simulink model "c00001M_harness"  (R2018a)
settings: Solver=ode3  StartTime=0.0  StopTime=10.0  RelTol=1e-3  EnableMultiTasking=on
undefined symbols (not defined in the file): b, DiscIntNeverNeededParam, J, K, L, R, sigbuilder_block
(part 3 of 19)

== system c00001M_harness/Eval66 ==
  In1 : Inport
  In2 : Inport  Port=2
  Constant3 : Constant
  Constant4 : Constant
  Data Type Conversion : DataTypeConversion
  Data Type Conversion1 : DataTypeConversion
  Memory1 : Memory  InitialCondition=1
  Memory2 : Memory  InitialCondition=1
  MinMax : MinMax  Inputs=4
  MinMax1 : MinMax  Inputs=2
  MinMax2 : MinMax  Inputs=2
  ROOut1 : RelationalOperator  Operator===  OutDataTypeStr=boolean  RndMeth=Simplest
  ROOut2 : RelationalOperator  Operator===  OutDataTypeStr=boolean  RndMeth=Simplest
  Out1 : Outport
  wires:
  Data Type Conversion1/1 -> MinMax2/1
  Data Type Conversion/1 -> MinMax1/1
  MinMax1/1 -> Memory1/1, MinMax/1
  MinMax2/1 -> Memory2/1, MinMax/2
  ROOut1/1 -> Data Type Conversion/1
  Memory2/1 -> MinMax2/2
  ROOut2/1 -> Data Type Conversion1/1
  Memory1/1 -> MinMax1/2
  [out2] -> ROOut2/2
  In1/1 -> ROOut1/1
  In2/1 -> ROOut2/1
  [out1] -> ROOut1/2
  MinMax/1 -> Out1/1
  Constant3/1 -> MinMax/3
  Constant4/1 -> MinMax/4

== system c00001M_harness/Eval67 ==
  In1 : Inport
  In2 : Inport  Port=2
  Constant3 : Constant
  Constant4 : Constant
  Data Type Conversion : DataTypeConversion
  Data Type Conversion1 : DataTypeConversion
  Memory1 : Memory  InitialCondition=1
  Memory2 : Memory  InitialCondition=1
  MinMax : MinMax  Inputs=4
  MinMax1 : MinMax  Inputs=2
  MinMax2 : MinMax  Inputs=2
  ROOut1 : RelationalOperator  Operator===  OutDataTypeStr=boolean  RndMeth=Simplest
  ROOut2 : RelationalOperator  Operator===  OutDataTypeStr=boolean  RndMeth=Simplest
  Out1 : Outport
  wires:
  Data Type Conversion1/1 -> MinMax2/1
  Data Type Conversion/1 -> MinMax1/1
  MinMax1/1 -> Memory1/1, MinMax/1
  MinMax2/1 -> Memory2/1, MinMax/2
  ROOut1/1 -> Data Type Conversion/1
  Memory2/1 -> MinMax2/2
  ROOut2/1 -> Data Type Conversion1/1
  Memory1/1 -> MinMax1/2
  [out2] -> ROOut2/2
  In1/1 -> ROOut1/1
  In2/1 -> ROOut2/1
  [out1] -> ROOut1/2
  MinMax/1 -> Out1/1
  Constant3/1 -> MinMax/3
  Constant4/1 -> MinMax/4

== system c00001M_harness/Eval70 ==
  In1 : Inport
  In2 : Inport  Port=2
  Constant3 : Constant
  Constant4 : Constant
  Data Type Conversion : DataTypeConversion
  Data Type Conversion1 : DataTypeConversion
  Memory1 : Memory  InitialCondition=1
  Memory2 : Memory  InitialCondition=1
  MinMax : MinMax  Inputs=4
  MinMax1 : MinMax  Inputs=2
  MinMax2 : MinMax  Inputs=2
  ROOut1 : RelationalOperator  Operator===  OutDataTypeStr=boolean  RndMeth=Simplest
  ROOut2 : RelationalOperator  Operator===  OutDataTypeStr=boolean  RndMeth=Simplest
  Out1 : Outport
  wires:
  Data Type Conversion1/1 -> MinMax2/1
  Data Type Conversion/1 -> MinMax1/1
  MinMax1/1 -> Memory1/1, MinMax/1
  MinMax2/1 -> Memory2/1, MinMax/2
  ROOut1/1 -> Data Type Conversion/1
  Memory2/1 -> MinMax2/2
  ROOut2/1 -> Data Type Conversion1/1
  Memory1/1 -> MinMax1/2
  [out2] -> ROOut2/2
  In1/1 -> ROOut1/1
  In2/1 -> ROOut2/1
  [out1] -> ROOut1/2
  MinMax/1 -> Out1/1
  Constant3/1 -> MinMax/3
  Constant4/1 -> MinMax/4

== system c00001M_harness/Eval71 ==
  In1 : Inport
  In2 : Inport  Port=2
  Constant3 : Constant
  Constant4 : Constant
  Data Type Conversion : DataTypeConversion
  Data Type Conversion1 : DataTypeConversion
  Memory1 : Memory  InitialCondition=1
  Memory2 : Memory  InitialCondition=1
  MinMax : MinMax  Inputs=4
  MinMax1 : MinMax  Inputs=2
  MinMax2 : MinMax  Inputs=2
  ROOut1 : RelationalOperator  Operator===  OutDataTypeStr=boolean  RndMeth=Simplest
  ROOut2 : RelationalOperator  Operator===  OutDataTypeStr=boolean  RndMeth=Simplest
  Out1 : Outport
  wires:
  Data Type Conversion1/1 -> MinMax2/1
  Data Type Conversion/1 -> MinMax1/1
  MinMax1/1 -> Memory1/1, MinMax/1
  MinMax2/1 -> Memory2/1, MinMax/2
  ROOut1/1 -> Data Type Conversion/1
  Memory2/1 -> MinMax2/2
  ROOut2/1 -> Data Type Conversion1/1
  Memory1/1 -> MinMax1/2
  [out2] -> ROOut2/2
  In1/1 -> ROOut1/1
  In2/1 -> ROOut2/1
  [out1] -> ROOut1/2
  MinMax/1 -> Out1/1
  Constant3/1 -> MinMax/3
  Constant4/1 -> MinMax/4

== system c00001M_harness/Eval74 ==
  In1 : Inport
  In2 : Inport  Port=2
  Constant3 : Constant
  Constant4 : Constant
  Data Type Conversion : DataTypeConversion
  Data Type Conversion1 : DataTypeConversion
  Memory1 : Memory  InitialCondition=1
  Memory2 : Memory  InitialCondition=1
  MinMax : MinMax  Inputs=4
  MinMax1 : MinMax  Inputs=2
  MinMax2 : MinMax  Inputs=2
  ROOut1 : RelationalOperator  Operator===  OutDataTypeStr=boolean  RndMeth=Simplest
  ROOut2 : RelationalOperator  Operator===  OutDataTypeStr=boolean  RndMeth=Simplest
  Out1 : Outport
  wires:
  Data Type Conversion1/1 -> MinMax2/1
  Data Type Conversion/1 -> MinMax1/1
  MinMax1/1 -> Memory1/1, MinMax/1
  MinMax2/1 -> Memory2/1, MinMax/2
  ROOut1/1 -> Data Type Conversion/1
  Memory2/1 -> MinMax2/2
  ROOut2/1 -> Data Type Conversion1/1
  Memory1/1 -> MinMax1/2
  [out2] -> ROOut2/2
  In1/1 -> ROOut1/1
  In2/1 -> ROOut2/1
  [out1] -> ROOut1/2
  MinMax/1 -> Out1/1
  Constant3/1 -> MinMax/3
  Constant4/1 -> MinMax/4

== system c00001M_harness/Eval75 ==
  In1 : Inport
  In2 : Inport  Port=2
  Constant3 : Constant
  Constant4 : Constant
  Data Type Conversion : DataTypeConversion
  Data Type Conversion1 : DataTypeConversion
  Memory1 : Memory  InitialCondition=1
  Memory2 : Memory  InitialCondition=1
  MinMax : MinMax  Inputs=4
  MinMax1 : MinMax  Inputs=2
  MinMax2 : MinMax  Inputs=2
  ROOut1 : RelationalOperator  Operator===  OutDataTypeStr=boolean  RndMeth=Simplest
  ROOut2 : RelationalOperator  Operator===  OutDataTypeStr=boolean  RndMeth=Simplest
  Out1 : Outport
  wires:
  Data Type Conversion1/1 -> MinMax2/1
  Data Type Conversion/1 -> MinMax1/1
  MinMax1/1 -> Memory1/1, MinMax/1
  MinMax2/1 -> Memory2/1, MinMax/2
  ROOut1/1 -> Data Type Conversion/1
  Memory2/1 -> MinMax2/2
  ROOut2/1 -> Data Type Conversion1/1
  Memory1/1 -> MinMax1/2
  [out2] -> ROOut2/2
  In1/1 -> ROOut1/1
  In2/1 -> ROOut2/1
  [out1] -> ROOut1/2
  MinMax/1 -> Out1/1
  Constant3/1 -> MinMax/3
  Constant4/1 -> MinMax/4

== system c00001M_harness/Eval78 ==
  In1 : Inport
  In2 : Inport  Port=2
  Constant3 : Constant
  Constant4 : Constant
  Data Type Conversion : DataTypeConversion
  Data Type Conversion1 : DataTypeConversion
  Memory1 : Memory  InitialCondition=1
  Memory2 : Memory  InitialCondition=1
  MinMax : MinMax  Inputs=4
  MinMax1 : MinMax  Inputs=2
  MinMax2 : MinMax  Inputs=2
  ROOut1 : RelationalOperator  Operator===  OutDataTypeStr=boolean  RndMeth=Simplest
  ROOut2 : RelationalOperator  Operator===  OutDataTypeStr=boolean  RndMeth=Simplest
  Out1 : Outport
  wires:
  Data Type Conversion1/1 -> MinMax2/1
  Data Type Conversion/1 -> MinMax1/1
  MinMax1/1 -> Memory1/1, MinMax/1
  MinMax2/1 -> Memory2/1, MinMax/2
  ROOut1/1 -> Data Type Conversion/1
  Memory2/1 -> MinMax2/2
  ROOut2/1 -> Data Type Conversion1/1
  Memory1/1 -> MinMax1/2
  [out2] -> ROOut2/2
  In1/1 -> ROOut1/1
  In2/1 -> ROOut2/1
  [out1] -> ROOut1/2
  MinMax/1 -> Out1/1
  Constant3/1 -> MinMax/3
  Constant4/1 -> MinMax/4

== system c00001M_harness/Eval79 ==
  In1 : Inport
  In2 : Inport  Port=2
  Constant3 : Constant
  Constant4 : Constant
  Data Type Conversion : DataTypeConversion
  Data Type Conversion1 : DataTypeConversion
  Memory1 : Memory  InitialCondition=1
  Memory2 : Memory  InitialCondition=1
  MinMax : MinMax  Inputs=4
  MinMax1 : MinMax  Inputs=2
  MinMax2 : MinMax  Inputs=2
  ROOut1 : RelationalOperator  Operator===  OutDataTypeStr=boolean  RndMeth=Simplest
  ROOut2 : RelationalOperator  Operator===  OutDataTypeStr=boolean  RndMeth=Simplest
  Out1 : Outport
  wires:
  Data Type Conversion1/1 -> MinMax2/1
  Data Type Conversion/1 -> MinMax1/1
  MinMax1/1 -> Memory1/1, MinMax/1
  MinMax2/1 -> Memory2/1, MinMax/2
  ROOut1/1 -> Data Type Conversion/1
  Memory2/1 -> MinMax2/2
  ROOut2/1 -> Data Type Conversion1/1
  Memory1/1 -> MinMax1/2
  [out2] -> ROOut2/2
  In1/1 -> ROOut1/1
  In2/1 -> ROOut2/1
  [out1] -> ROOut1/2
  MinMax/1 -> Out1/1
  Constant3/1 -> MinMax/3
  Constant4/1 -> MinMax/4

== system c00001M_harness/Eval82 ==
  In1 : Inport
  In2 : Inport  Port=2
  Constant3 : Constant
  Constant4 : Constant
  Data Type Conversion : DataTypeConversion
  Data Type Conversion1 : DataTypeConversion
  Memory1 : Memory  InitialCondition=1
  Memory2 : Memory  InitialCondition=1
  MinMax : MinMax  Inputs=4
  MinMax1 : MinMax  Inputs=2
  MinMax2 : MinMax  Inputs=2
  ROOut1 : RelationalOperator  Operator===  OutDataTypeStr=boolean  RndMeth=Simplest
  ROOut2 : RelationalOperator  Operator===  OutDataTypeStr=boolean  RndMeth=Simplest
  Out1 : Outport
  wires:
  Data Type Conversion1/1 -> MinMax2/1
  Data Type Conversion/1 -> MinMax1/1
  MinMax1/1 -> Memory1/1, MinMax/1
  MinMax2/1 -> Memory2/1, MinMax/2
  ROOut1/1 -> Data Type Conversion/1
  Memory2/1 -> MinMax2/2
  ROOut2/1 -> Data Type Conversion1/1
  Memory1/1 -> MinMax1/2
  [out2] -> ROOut2/2
  In1/1 -> ROOut1/1
  In2/1 -> ROOut2/1
  [out1] -> ROOut1/2
  MinMax/1 -> Out1/1
  Constant3/1 -> MinMax/3
  Constant4/1 -> MinMax/4

== system c00001M_harness/Eval83 ==
  In1 : Inport
  In2 : Inport  Port=2
  Constant3 : Constant
  Constant4 : Constant
  Data Type Conversion : DataTypeConversion
  Data Type Conversion1 : DataTypeConversion
  Memory1 : Memory  InitialCondition=1
  Memory2 : Memory  InitialCondition=1
  MinMax : MinMax  Inputs=4
  MinMax1 : MinMax  Inputs=2
  MinMax2 : MinMax  Inputs=2
  ROOut1 : RelationalOperator  Operator===  OutDataTypeStr=boolean  RndMeth=Simplest
  ROOut2 : RelationalOperator  Operator===  OutDataTypeStr=boolean  RndMeth=Simplest
  Out1 : Outport
  wires:
  Data Type Conversion1/1 -> MinMax2/1
  Data Type Conversion/1 -> MinMax1/1
  MinMax1/1 -> Memory1/1, MinMax/1
  MinMax2/1 -> Memory2/1, MinMax/2
  ROOut1/1 -> Data Type Conversion/1
  Memory2/1 -> MinMax2/2
  ROOut2/1 -> Data Type Conversion1/1
  Memory1/1 -> MinMax1/2
  [out2] -> ROOut2/2
  In1/1 -> ROOut1/1
  In2/1 -> ROOut2/1
  [out1] -> ROOut1/2
  MinMax/1 -> Out1/1
  Constant3/1 -> MinMax/3
  Constant4/1 -> MinMax/4

== system c00001M_harness/Eval86 ==
  In1 : Inport
  In2 : Inport  Port=2
  Constant3 : Constant
  Constant4 : Constant
  Data Type Conversion : DataTypeConversion
  Data Type Conversion1 : DataTypeConversion
  Memory1 : Memory  InitialCondition=1
  Memory2 : Memory  InitialCondition=1
  MinMax : MinMax  Inputs=4
  MinMax1 : MinMax  Inputs=2
  MinMax2 : MinMax  Inputs=2
  ROOut1 : RelationalOperator  Operator===  OutDataTypeStr=boolean  RndMeth=Simplest
  ROOut2 : RelationalOperator  Operator===  OutDataTypeStr=boolean  RndMeth=Simplest
  Out1 : Outport
  wires:
  Data Type Conversion1/1 -> MinMax2/1
  Data Type Conversion/1 -> MinMax1/1
  MinMax1/1 -> Memory1/1, MinMax/1
  MinMax2/1 -> Memory2/1, MinMax/2
  ROOut1/1 -> Data Type Conversion/1
  Memory2/1 -> MinMax2/2
  ROOut2/1 -> Data Type Conversion1/1
  Memory1/1 -> MinMax1/2
  [out2] -> ROOut2/2
  In1/1 -> ROOut1/1
  In2/1 -> ROOut2/1
  [out1] -> ROOut1/2
  MinMax/1 -> Out1/1
  Constant3/1 -> MinMax/3
  Constant4/1 -> MinMax/4

== system c00001M_harness/Eval87 ==
  In1 : Inport
  In2 : Inport  Port=2
  Constant3 : Constant
  Constant4 : Constant
  Data Type Conversion : DataTypeConversion
  Data Type Conversion1 : DataTypeConversion
  Memory1 : Memory  InitialCondition=1
  Memory2 : Memory  InitialCondition=1
  MinMax : MinMax  Inputs=4
  MinMax1 : MinMax  Inputs=2
  MinMax2 : MinMax  Inputs=2
  ROOut1 : RelationalOperator  Operator===  OutDataTypeStr=boolean  RndMeth=Simplest
  ROOut2 : RelationalOperator  Operator===  OutDataTypeStr=boolean  RndMeth=Simplest
  Out1 : Outport
  wires:
  Data Type Conversion1/1 -> MinMax2/1
  Data Type Conversion/1 -> MinMax1/1
  MinMax1/1 -> Memory1/1, MinMax/1
  MinMax2/1 -> Memory2/1, MinMax/2
  ROOut1/1 -> Data Type Conversion/1
  Memory2/1 -> MinMax2/2
  ROOut2/1 -> Data Type Conversion1/1
  Memory1/1 -> MinMax1/2
  [out2] -> ROOut2/2
  In1/1 -> ROOut1/1
  In2/1 -> ROOut2/1
  [out1] -> ROOut1/2
  MinMax/1 -> Out1/1
  Constant3/1 -> MinMax/3
  Constant4/1 -> MinMax/4

== system c00001M_harness/Eval90 ==
  In1 : Inport
  In2 : Inport  Port=2
  Constant3 : Constant
  Constant4 : Constant
  Data Type Conversion : DataTypeConversion
  Data Type Conversion1 : DataTypeConversion
  Memory1 : Memory  InitialCondition=1
  Memory2 : Memory  InitialCondition=1
  MinMax : MinMax  Inputs=4
  MinMax1 : MinMax  Inputs=2
  MinMax2 : MinMax  Inputs=2
  ROOut1 : RelationalOperator  Operator===  OutDataTypeStr=boolean  RndMeth=Simplest
  ROOut2 : RelationalOperator  Operator===  OutDataTypeStr=boolean  RndMeth=Simplest
  Out1 : Outport
  wires:
  Data Type Conversion1/1 -> MinMax2/1
  Data Type Conversion/1 -> MinMax1/1
  MinMax1/1 -> Memory1/1, MinMax/1
  MinMax2/1 -> Memory2/1, MinMax/2
  ROOut1/1 -> Data Type Conversion/1
  Memory2/1 -> MinMax2/2
  ROOut2/1 -> Data Type Conversion1/1
  Memory1/1 -> MinMax1/2
  [out2] -> ROOut2/2
  In1/1 -> ROOut1/1
  In2/1 -> ROOut2/1
  [out1] -> ROOut1/2
  MinMax/1 -> Out1/1
  Constant3/1 -> MinMax/3
  Constant4/1 -> MinMax/4

== system c00001M_harness/Eval91 ==
  In1 : Inport
  In2 : Inport  Port=2
  Constant3 : Constant
  Constant4 : Constant
  Data Type Conversion : DataTypeConversion
  Data Type Conversion1 : DataTypeConversion
  Memory1 : Memory  InitialCondition=1
  Memory2 : Memory  InitialCondition=1
  MinMax : MinMax  Inputs=4
  MinMax1 : MinMax  Inputs=2
  MinMax2 : MinMax  Inputs=2
  ROOut1 : RelationalOperator  Operator===  OutDataTypeStr=boolean  RndMeth=Simplest
  ROOut2 : RelationalOperator  Operator===  OutDataTypeStr=boolean  RndMeth=Simplest
  Out1 : Outport
  wires:
  Data Type Conversion1/1 -> MinMax2/1
  Data Type Conversion/1 -> MinMax1/1
  MinMax1/1 -> Memory1/1, MinMax/1
  MinMax2/1 -> Memory2/1, MinMax/2
  ROOut1/1 -> Data Type Conversion/1
  Memory2/1 -> MinMax2/2
  ROOut2/1 -> Data Type Conversion1/1
  Memory1/1 -> MinMax1/2
  [out2] -> ROOut2/2
  In1/1 -> ROOut1/1
  In2/1 -> ROOut2/1
  [out1] -> ROOut1/2
  MinMax/1 -> Out1/1
  Constant3/1 -> MinMax/3
  Constant4/1 -> MinMax/4

== system c00001M_harness/Eval94 ==
  In1 : Inport
  In2 : Inport  Port=2
  Constant3 : Constant
  Constant4 : Constant
  Data Type Conversion : DataTypeConversion
  Data Type Conversion1 : DataTypeConversion
  Memory1 : Memory  InitialCondition=1
  Memory2 : Memory  InitialCondition=1
  MinMax : MinMax  Inputs=4
  MinMax1 : MinMax  Inputs=2
  MinMax2 : MinMax  Inputs=2
  ROOut1 : RelationalOperator  Operator===  OutDataTypeStr=boolean  RndMeth=Simplest
  ROOut2 : RelationalOperator  Operator===  OutDataTypeStr=boolean  RndMeth=Simplest
  Out1 : Outport
  wires:
  Data Type Conversion1/1 -> MinMax2/1
  Data Type Conversion/1 -> MinMax1/1
  MinMax1/1 -> Memory1/1, MinMax/1
  MinMax2/1 -> Memory2/1, MinMax/2
  ROOut1/1 -> Data Type Conversion/1
  Memory2/1 -> MinMax2/2
  ROOut2/1 -> Data Type Conversion1/1
  Memory1/1 -> MinMax1/2
  [out2] -> ROOut2/2
  In1/1 -> ROOut1/1
  In2/1 -> ROOut2/1
  [out1] -> ROOut1/2
  MinMax/1 -> Out1/1
  Constant3/1 -> MinMax/3
  Constant4/1 -> MinMax/4

== system c00001M_harness/Eval95 ==
  In1 : Inport
  In2 : Inport  Port=2
  Constant3 : Constant
  Constant4 : Constant
  Data Type Conversion : DataTypeConversion
  Data Type Conversion1 : DataTypeConversion
  Memory1 : Memory  InitialCondition=1
  Memory2 : Memory  InitialCondition=1
  MinMax : MinMax  Inputs=4
  MinMax1 : MinMax  Inputs=2
  MinMax2 : MinMax  Inputs=2
  ROOut1 : RelationalOperator  Operator===  OutDataTypeStr=boolean  RndMeth=Simplest
  ROOut2 : RelationalOperator  Operator===  OutDataTypeStr=boolean  RndMeth=Simplest
  Out1 : Outport
  wires:
  Data Type Conversion1/1 -> MinMax2/1
  Data Type Conversion/1 -> MinMax1/1
  MinMax1/1 -> Memory1/1, MinMax/1
  MinMax2/1 -> Memory2/1, MinMax/2
  ROOut1/1 -> Data Type Conversion/1
  Memory2/1 -> MinMax2/2
  ROOut2/1 -> Data Type Conversion1/1
  Memory1/1 -> MinMax1/2
  [out2] -> ROOut2/2
  In1/1 -> ROOut1/1
  In2/1 -> ROOut2/1
  [out1] -> ROOut1/2
  MinMax/1 -> Out1/1
  Constant3/1 -> MinMax/3
  Constant4/1 -> MinMax/4

== system c00001M_harness/Eval98 ==
  In1 : Inport
  In2 : Inport  Port=2
  Constant3 : Constant
  Constant4 : Constant
  Data Type Conversion : DataTypeConversion
  Data Type Conversion1 : DataTypeConversion
  Memory1 : Memory  InitialCondition=1
  Memory2 : Memory  InitialCondition=1
  MinMax : MinMax  Inputs=4
  MinMax1 : MinMax  Inputs=2
  MinMax2 : MinMax  Inputs=2
  ROOut1 : RelationalOperator  Operator===  OutDataTypeStr=boolean  RndMeth=Simplest
  ROOut2 : RelationalOperator  Operator===  OutDataTypeStr=boolean  RndMeth=Simplest
  Out1 : Outport
  wires:
  Data Type Conversion1/1 -> MinMax2/1
  Data Type Conversion/1 -> MinMax1/1
  MinMax1/1 -> Memory1/1, MinMax/1
  MinMax2/1 -> Memory2/1, MinMax/2
  ROOut1/1 -> Data Type Conversion/1
  Memory2/1 -> MinMax2/2
  ROOut2/1 -> Data Type Conversion1/1
  Memory1/1 -> MinMax1/2
  [out2] -> ROOut2/2
  In1/1 -> ROOut1/1
  In2/1 -> ROOut2/1
  [out1] -> ROOut1/2
  MinMax/1 -> Out1/1
  Constant3/1 -> MinMax/3
  Constant4/1 -> MinMax/4

== system c00001M_harness/Eval99 ==
  In1 : Inport
  In2 : Inport  Port=2
  Constant3 : Constant
  Constant4 : Constant
  Data Type Conversion : DataTypeConversion
  Data Type Conversion1 : DataTypeConversion
  Memory1 : Memory  InitialCondition=1
  Memory2 : Memory  InitialCondition=1
  MinMax : MinMax  Inputs=4
  MinMax1 : MinMax  Inputs=2
  MinMax2 : MinMax  Inputs=2
  ROOut1 : RelationalOperator  Operator===  OutDataTypeStr=boolean  RndMeth=Simplest
  ROOut2 : RelationalOperator  Operator===  OutDataTypeStr=boolean  RndMeth=Simplest
  Out1 : Outport
  wires:
  Data Type Conversion1/1 -> MinMax2/1
  Data Type Conversion/1 -> MinMax1/1
  MinMax1/1 -> Memory1/1, MinMax/1
  MinMax2/1 -> Memory2/1, MinMax/2
  ROOut1/1 -> Data Type Conversion/1
  Memory2/1 -> MinMax2/2
  ROOut2/1 -> Data Type Conversion1/1
  Memory1/1 -> MinMax1/2
  [out2] -> ROOut2/2
  In1/1 -> ROOut1/1
  In2/1 -> ROOut2/1
  [out1] -> ROOut1/2
  MinMax/1 -> Out1/1
  Constant3/1 -> MinMax/3
  Constant4/1 -> MinMax/4

== system c00001M_harness/Inputs ==
  Demux : Demux  Tag=STV Demux
  FromWs : FromWorkspace  Tag=STV FromWs  VariableName=tuvar  SampleTime=0
      SigBuilderData=|
      | dataSet(1).timeRange = [0 20]
      | dataSet(1).name = 'Test Case 1'
      | dataSet(2).timeRange = [0 10]
      | dataSet(2).name = 'Test Case 2'
      | dataSet(3).timeRange = [0 8]
      | dataSet(3).name = 'Test Case 3'
      | dataSet(4).timeRange = [0 6]
      | dataSet(4).name = 'Test Case 4'
      | dataSet(5).timeRange = [0 6]
      | dataSet(5).name = 'Test Case 5'
      | dataSet(6).timeRange = [0 6]
      | dataSet(6).name = 'Test Case 6'
      | dataSet(7).timeRange = [0 8]
      | dataSet(7).name = 'Test Case 7'
      | dataSet(8).timeRange = [0 6]
      | dataSet(8).name = 'Test Case 8'
      | dataSet(9).timeRange = [0 6]
      | dataSet(9).name = 'Test Case 9'
      | dataSet(10).timeRange = [0 7]
      | dataSet(10).name = 'Test Case 10'
      | dataSet(11).timeRange = [0 9]
      | dataSet(11).name = 'Test Case 11'
      | dataSet(12).timeRange = [0 8]
      | dataSet(12).name = 'Test Case 12'
      | dataSet(13).timeRange = [0 12]
      | dataSet(13).name = 'Test Case 13'
      | dataSet(14).timeRange = [0 8]
      | dataSet(14).name = 'Test Case 14'
      | dataSet(15).timeRange = [0 8]
      | dataSet(15).name = 'Test Case 15'
      | dataSet(16).timeRange = [0 8]
      | dataSet(16).name = 'Test Case 16'
      | dataSet(17).timeRange = [0 8]
      | dataSet(17).name = 'Test Case 17'
      | dataSet(18).timeRange = [0 8]
      | dataSet(18).name = 'Test Case 18'
      | dataSet(19).timeRange = [0 8]
      | dataSet(19).name = 'Test Case 19'
      | dataSet(20).timeRange = [0 7]
      | dataSet(20).name = 'Test Case 20'
      | dataSet(21).timeRange = [0 7]
      | dataSet(21).name = 'Test Case 21'
      | dataSet(22).timeRange = [0 7]
      | dataSet(22).name = 'Test Case 22'
      | dataSet(23).timeRange = [0 8]
      | dataSet(23).name = 'Test Case 23'
      | dataSet(24).timeRange = [0 8]
      | dataSet(24).name = 'Test Case 24'
      | dataSet(25).timeRange = [0 8]
      | dataSet(25).name = 'Test Case 25'
      | dataSet(26).timeRange = [0 8]
      | dataSet(26).name = 'Test Case 26'
      | sbobj.Name = 'Signal Builder'
      | sbobj.Groups(1).Name = 'Test Case 1'
      | sbobj.Groups(1).Signals(1).Name = 'DW1'
      | sbobj.Groups(1).Signals(1).XData = [0 2 8 11 11 13 16 17 17 19 19 20]
      | sbobj.Groups(1).Signals(1).YData = [1 1 1 1 0 0 0 0 4 4 3 3]
      | sbobj.Groups(1).Signals(2).Name = 'P1W2'
      | sbobj.Groups(1).Signals(2).XData = [0 2 2 8 8 11 11 13 13 16 16 17 17 19 19 20]
      | sbobj.Groups(1).Signals(2).YData = [2 2 2 2 4 4 3 3 1 1 0 0 0 0 0 0]
      | sbobj.Groups(1).Signals(3).Name = 'O1'
      | sbobj.Groups(1).Signals(3).XData = [0 2 2 8 8 11 11 13 13 16 16 17 17 19 19 20]
      | sbobj.Groups(1).Signals(3).YData = [1 1 1 1 1 1 1 1 1 1 0 0 0 0 0 0]
      | sbobj.Groups(1).Signals(4).Name = 'O2'
      | sbobj.Groups(1).Signals(4).XData = [0 2 2 8 8 11 11 13 13 16 16 17 17 19 19 20]
      | sbobj.Groups(1).Signals(4).YData = [0 0 1 1 0 0 0 0 0 0 0 0 0 0 0 0]
      | sbobj.Groups(1).TimeRange = [0 20]
      | sbobj.Groups(2).Name = 'Test Case 2'
      | sbobj.Groups(2).Signals(1).Name = 'DW1'
      | sbobj.Groups(2).Signals(1).XData = [0 3 3 5 5 9 9 10]
      | sbobj.Groups(2).Signals(1).YData = [3 3 3 3 2 2 2 2]
      | sbobj.Groups(2).Signals(2).Name = 'P1W2'
      | sbobj.Groups(2).Signals(2).XData = [0 3 3 5 5 9 9 10]
      | sbobj.Groups(2).Signals(2).YData = [3 3 0 0 0 0 1 1]
      | sbobj.Groups(2).Signals(3).Name = 'O1'
      | sbobj.Groups(2).Signals(3).XData = [0 3 3 5 5 9 9 10]
      | sbobj.Groups(2).Signals(3).YData = [1 1 1 1 0 0 0 0]
      | sbobj.Groups(2).Signals(4).Name = 'O2'
      | sbobj.Groups(2).Signals(4).XData = [0 3 3 5 5 9 9 10]
      | sbobj.Groups(2).Signals(4).YData = [0 0 0 0 0 0 0 0]
      | sbobj.Groups(3).Name = 'Test Case 3'
      | sbobj.Groups(3).Signals(1).Name = 'DW1'
      | sbobj.Groups(3).Signals(1).XData = [0 3 3 4 4 7 7 8]
      | sbobj.Groups(3).Signals(1).YData = [4 4 0 0 1 1 1 1]
      | sbobj.Groups(3).Signals(2).Name = 'P1W2'
      | sbobj.Groups(3).Signals(2).XData = [0 3 3 4 4 7 7 8]
      | sbobj.Groups(3).Signals(2).YData = [4 4 1 1 0 0 3 3]
      | sbobj.Groups(3).Signals(3).Name = 'O1'
      | sbobj.Groups(3).Signals(3).XData = [0 3 3 4 4 7 7 8]
      | sbobj.Groups(3).Signals(3).YData = [0 0 0 0 0 0 0 0]
      | sbobj.Groups(3).Signals(4).Name = 'O2'
      | sbobj.Groups(3).Signals(4).XData = [0 3 3 4 4 7 7 8]
      | sbobj.Groups(3).Signals(4).YData = [0 0 0 0 0 0 0 0]
      | sbobj.Groups(3).TimeRange = [0 8]
      | sbobj.Groups(4).Name = 'Test Case 4'
      | sbobj.Groups(4).Signals(1).Name = 'DW1'
      | sbobj.Groups(4).Signals(1).XData = [0 3 3 5 5 6]
      | sbobj.Groups(4).Signals(1).YData = [4 4 2 2 2 2]
      | sbobj.Groups(4).Signals(2).Name = 'P1W2'
      | sbobj.Groups(4).Signals(2).XData = [0 3 3 5 5 6]
      | sbobj.Groups(4).Signals(2).YData = [1 1 0 0 0 0]
      | sbobj.Groups(4).Signals(3).Name = 'O1'
      | sbobj.Groups(4).Signals(3).XData = [0 3 3 5 5 6]
      | sbobj.Groups(4).Signals(3).YData = [0 0 0 0 0 0]
      | sbobj.Groups(4).Signals(4).Name = 'O2'
      | sbobj.Groups(4).Signals(4).XData = [0 3 3 5 5 6]
      | sbobj.Groups(4).Signals(4).YData = [0 0 0 0 1 1]
      | sbobj.Groups(4).TimeRange = [0 6]
      | sbobj.Groups(5).Name = 'Test Case 5'
      | sbobj.Groups(5).Signals(1).Name = 'DW1'
      | sbobj.Groups(5).Signals(1).XData = [0 3 3 5 5 6]
      | sbobj.Groups(5).Signals(1).YData = [3 3 0 0 3 3]
      | sbobj.Groups(5).Signals(2).Name = 'P1W2'
      | sbobj.Groups(5).Signals(2).XData = [0 3 3 5 5 6]
      | sbobj.Groups(5).Signals(2).YData = [4 4 0 0 3 3]
      | sbobj.Groups(5).Signals(3).Name = 'O1'
      | sbobj.Groups(5).Signals(3).XData = [0 3 3 5 5 6]
      | sbobj.Groups(5).Signals(3).YData = [0 0 0 0 1 1]
      | sbobj.Groups(5).Signals(4).Name = 'O2'
      | sbobj.Groups(5).Signals(4).XData = [0 3 3 5 5 6]
      | sbobj.Groups(5).Signals(4).YData = [1 1 0 0 0 0]
      | sbobj.Groups(5).TimeRange = [0 6]
      | sbobj.Groups(6).Name = 'Test Case 6'
      | sbobj.Groups(6).Signals(1).Name = 'DW1'
      | sbobj.Groups(6).Signals(1).XData = [0 3 3 5 5 6]
      | sbobj.Groups(6).Signals(1).YData = [1 1 1 1 0 0]
      | sbobj.Groups(6).Signals(2).Name = 'P1W2'
      | sbobj.Groups(6).Signals(2).XData = [0 3 3 5 5 6]
      | sbobj.Groups(6).Signals(2).YData = [4 4 2 2 0 0]
      | sbobj.Groups(6).Signals(3).Name = 'O1'
      | sbobj.Groups(6).Signals(3).XData = [0 3 3 5 5 6]
      | sbobj.Groups(6).Signals(3).YData = [1 1 1 1 1 1]
      | sbobj.Groups(6).Signals(4).Name = 'O2'
      | sbobj.Groups(6).Signals(4).XData = [0 3 3 5 5 6]
      | sbobj.Groups(6).Signals(4).YData = [0 0 0 0 1 1]
      | sbobj.Groups(6).TimeRange = [0 6]
      | sbobj.Groups(7).Name = 'Test Case 7'
      | sbobj.Groups(7).Signals(1).Name = 'DW1'
      | sbobj.Groups(7).Signals(1).XData = [0 3 3 4 4 7 7 8]
      | sbobj.Groups(7).Signals(1).YData = [1 1 1 1 1 1 3 3]
      | sbobj.Groups(7).Signals(2).Name = 'P1W2'
      | sbobj.Groups(7).Signals(2).XData = [0 3 3 4 4 7 7 8]
      | sbobj.Groups(7).Signals(2).YData = [4 4 3 3 2 2 0 0]
      | sbobj.Groups(7).Signals(3).Name = 'O1'
      | sbobj.Groups(7).Signals(3).XData = [0 3 3 4 4 7 7 8]
      | sbobj.Groups(7).Signals(3).YData = [1 1 1 1 1 1 0 0]
      | sbobj.Groups(7).Signals(4).Name = 'O2'
      | sbobj.Groups(7).Signals(4).XData = [0 3 3 4 4 7 7 8]
      | sbobj.Groups(7).Signals(4).YData = [0 0 0 0 0 0 1 1]
      | sbobj.Groups(7).TimeRange = [0 8]
      | sbobj.Groups(8).Name = 'Test Case 8'
      | sbobj.Groups(8).Signals(1).Name = 'DW1'
      | sbobj.Groups(8).Signals(1).XData = [0 2 2 3 3 5 5 6]
      | sbobj.Groups(8).Signals(1).YData = [1 1 2 2 2 2 2 2]
      | sbobj.Groups(8).Signals(2).Name = 'P1W2'
      | sbobj.Groups(8).Signals(2).XData = [0 2 2 3 3 5 5 6]
      | sbobj.Groups(8).Signals(2).YData = [4 4 3 3 1 1 3 3]
      | sbobj.Groups(8).Signals(3).Name = 'O1'
      | sbobj.Groups(8).Signals(3).XData = [0 2 2 3 3 5 5 6]
      | sbobj.Groups(8).Signals(3).YData = [1 1 1 1 1 1 0 0]
      | sbobj.Groups(8).Signals(4).Name = 'O2'
      | sbobj.Groups(8).Signals(4).XData = [0 2 2 3 3 5 5 6]
      | sbobj.Groups(8).Signals(4).YData = [0 0 1 1 0 0 0 0]
      | sbobj.Groups(8).TimeRange = [0 6]
      | sbobj.Groups(9).Name = 'Test Case 9'
      | sbobj.Groups(9).Signals(1).Name = 'DW1'
      | sbobj.Groups(9).Signals(1).XData = [0 2 2 3 3 5 5 6]
      | sbobj.Groups(9).Signals(1).YData = [1 1 4 4 3 3 2 2]
      | sbobj.Groups(9).Signals(2).Name = 'P1W2'
      | sbobj.Groups(9).Signals(2).XData = [0 2 2 3 3 5 5 6]
      | sbobj.Groups(9).Signals(2).YData = [4 4 0 0 0 0 1 1]
      | sbobj.Groups(9).Signals(3).Name = 'O1'
      | sbobj.Groups(9).Signals(3).XData = [0 2 2 3 3 5 5 6]
      | sbobj.Groups(9).Signals(3).YData = [1 1 1 1 0 0 1 1]
      | sbobj.Groups(9).Signals(4).Name = 'O2'
      | sbobj.Groups(9).Signals(4).XData = [0 2 2 3 3 5 5 6]
      | sbobj.Groups(9).Signals(4).YData = [0 0 1 1 0 0 1 1]
      | sbobj.Groups(9).TimeRange = [0 6]
      | sbobj.Groups(10).Name = 'Test Case 10'
      | sbobj.Groups(10).Signals(1).Name = 'DW1'
      | sbobj.Groups(10).Signals(1).XData = [0 2 2 3 3 6 6 7]
      | sbobj.Groups(10).Signals(1).YData = [1 1 3 3 2 2 0 0]
      | sbobj.Groups(10).Signals(2).Name = 'P1W2'
      | sbobj.Groups(10).Signals(2).XData = [0 2 2 3 3 6 6 7]
      | sbobj.Groups(10).Signals(2).YData = [4 4 0 0 0 0 1 1]
      | sbobj.Groups(10).Signals(3).Name = 'O1'
      | sbobj.Groups(10).Signals(3).XData = [0 2 2 3 3 6 6 7]
      | sbobj.Groups(10).Signals(3).YData = [1 1 1 1 0 0 0 0]
      | sbobj.Groups(10).Signals(4).Name = 'O2'
      | sbobj.Groups(10).Signals(4).XData = [0 2 2 3 3 6 6 7]
      | sbobj.Groups(10).Signals(4).YData = [0 0 1 1 0 0 0 0]
      | sbobj.Groups(10).TimeRange = [0 7]
      | sbobj.Groups(11).Name = 'Test Case 11'
      | sbobj.Groups(11).Signals(1).Name = 'DW1'
      | sbobj.Groups(11).Signals(1).XData = [0 4 4 5 5 7 7 8 8 9]
      | sbobj.Groups(11).Signals(1).YData = [3 3 1 1 0 0 2 2 3 3]
      | sbobj.Groups(11).Signals(2).Name = 'P1W2'
      | sbobj.Groups(11).Signals(2).XData = [0 4 4 5 5 7 7 8 8 9]
      | sbobj.Groups(11).Signals(2).YData = [4 4 0 0 0 0 2 2 3 3]
      | sbobj.Groups(11).Signals(3).Name = 'O1'
      | sbobj.Groups(11).Signals(3).XData = [0 4 4 5 5 7 7 8 8 9]
      | sbobj.Groups(11).Signals(3).YData = [0 0 0 0 0 0 0 0 1 1]
      | sbobj.Groups(11).Signals(4).Name = 'O2'
      | sbobj.Groups(11).Signals(4).XData = [0 4 4 5 5 7 7 8 8 9]
      | sbobj.Groups(11).Signals(4).YData = [1 1 0 0 0 0 0 0 1 1]
      | sbobj.Groups(11).TimeRange = [0 9]
      | sbobj.Groups(12).Name = 'Test Case 12'
      | sbobj.Groups(12).Signals(1).Name = 'DW1'
      | sbobj.Groups(12).Signals(1).XData = [0 4 4 6 6 7 7 8]
      | sbobj.Groups(12).Signals(1).YData = [3 3 4 4 1 1 3 3]
      | sbobj.Groups(12).Signals(2).Name = 'P1W2'
      | sbobj.Groups(12).Signals(2).XData = [0 4 4 6 6 7 7 8]
      | sbobj.Groups(12).Signals(2).YData = [4 4 0 0 1 1 2 2]
      | sbobj.Groups(12).Signals(3).Name = 'O1'
      | sbobj.Groups(12).Signals(3).XData = [0 4 4 6 6 7 7 8]
      | sbobj.Groups(12).Signals(3).YData = [0 0 0 0 1 1 0 0]
      | sbobj.Groups(12).Signals(4).Name = 'O2'
      | sbobj.Groups(12).Signals(4).XData = [0 4 4 6 6 7 7 8]
      | sbobj.Groups(12).Signals(4).YData = [1 1 0 0 0 0 1 1]
      | sbobj.Groups(12).TimeRange = [0 8]
      | sbobj.Groups(13).Name = 'Test Case 13'
      | sbobj.Groups(13).Signals(1).Name = 'DW1'
      | sbobj.Groups(13).Signals(1).XData = [0 2 2 3 3 5 5 6 6 8 8 11 11 12]
      | sbobj.Groups(13).Signals(1).YData = [4 4 4 4 0 0 1 1 1 1 4 4 2 2]
      | sbobj.Groups(13).Signals(2).Name = 'P1W2'
      | sbobj.Groups(13).Signals(2).XData = [0 2 2 3 3 5 5 6 6 8 8 11 11 12]
      | sbobj.Groups(13).Signals(2).YData = [1 1 3 3 4 4 2 2 3 3 0 0 1 1]
      | sbobj.Groups(13).Signals(3).Name = 'O1'
      | sbobj.Groups(13).Signals(3).XData = [0 2 2 3 3 5 5 6 6 8 8 11 11 12]
      | sbobj.Groups(13).Signals(3).YData = [0 0 1 1 1 1 1 1 1 1 1 1 0 0]
      | sbobj.Groups(13).Signals(4).Name = 'O2'
      | sbobj.Groups(13).Signals(4).XData = [0 2 2 3 3 5 5 6 6 8 8 11 11 12]
      | sbobj.Groups(13).Signals(4).YData = [0 0 1 1 0 0 0 0 0 0 0 0 1 1]
      | sbobj.Groups(13).TimeRange = [0 12]
      | sbobj.Groups(14).Name = 'Test Case 14'
      | sbobj.Groups(14).Signals(1).Name = 'DW1'
      | sbobj.Groups(14).Signals(1).XData = [0 3 3 4 4 5 5 7 7 8]
      | sbobj.Groups(14).Signals(1).YData = [4 4 0 0 1 1 4 4 3 3]
      | sbobj.Groups(14).Signals(2).Name = 'P1W2'
      | sbobj.Groups(14).Signals(2).XData = [0 3 3 4 4 5 5 7 7 8]
      | sbobj.Groups(14).Signals(2).YData = [4 4 1 1 0 0 0 0 2 2]
      | sbobj.Groups(14).Signals(3).Name = 'O1'
      | sbobj.Groups(14).Signals(3).XData = [0 3 3 4 4 5 5 7 7 8]
      | sbobj.Groups(14).Signals(3).YData = [0 0 0 0 0 0 0 0 0 0]
      | sbobj.Groups(14).Signals(4).Name = 'O2'
      | sbobj.Groups(14).Signals(4).XData = [0 3 3 4 4 5 5 7 7 8]
      | sbobj.Groups(14).Signals(4).YData = [0 0 0 0 0 0 0 0 1 1]
      | sbobj.Groups(14).TimeRange = [0 8]
      | sbobj.Groups(15).Name = 'Test Case 15'
      | sbobj.Groups(15).Signals(1).Name = 'DW1'
      | sbobj.Groups(15).Signals(1).XData = [0 3 3 4 4 5 5 7 7 8]
      | sbobj.Groups(15).Signals(1).YData = [4 4 0 0 1 1 3 3 0 0]
      | sbobj.Groups(15).Signals(2).Name = 'P1W2'
      | sbobj.Groups(15).Signals(2).XData = [0 3 3 4 4 5 5 7 7 8]
      | sbobj.Groups(15).Signals(2).YData = [4 4 1 1 0 0 0 0 0 0]
      | sbobj.Groups(15).Signals(3).Name = 'O1'
      | sbobj.Groups(15).Signals(3).XData = [0 3 3 4 4 5 5 7 7 8]
      | sbobj.Groups(15).Signals(3).YData = [0 0 0 0 0 0 0 0 1 1]
      | sbobj.Groups(15).Signals(4).Name = 'O2'
      | sbobj.Groups(15).Signals(4).XData = [0 3 3 4 4 5 5 7 7 8]
      | sbobj.Groups(15).Signals(4).YData = [0 0 0 0 0 0 0 0 1 1]
      | sbobj.Groups(15).TimeRange = [0 8]
      | sbobj.Groups(16).Name = 'Test Case 16'
      | sbobj.Groups(16).Signals(1).Name = 'DW1'
      | sbobj.Groups(16).Signals(1).XData = [0 3 3 4 4 5 5 7 7 8]
      | sbobj.Groups(16).Signals(1).YData = [4 4 0 0 1 1 2 2 3 3]
      | sbobj.Groups(16).Signals(2).Name = 'P1W2'
      | sbobj.Groups(16).Signals(2).XData = [0 3 3 4 4 5 5 7 7 8]
      | sbobj.Groups(16).Signals(2).YData = [4 4 1 1 0 0 0 0 4 4]
      | sbobj.Groups(16).Signals(3).Name = 'O1'
      | sbobj.Groups(16).Signals(3).XData = [0 3 3 4 4 5 5 7 7 8]
      | sbobj.Groups(16).Signals(3).YData = [0 0 0 0 0 0 0 0 0 0]
      | sbobj.Groups(16).Signals(4).Name = 'O2'
      | sbobj.Groups(16).Signals(4).XData = [0 3 3 4 4 5 5 7 7 8]
      | sbobj.Groups(16).Signals(4).YData = [0 0 0 0 0 0 0 0 1 1]
      | sbobj.Groups(16).TimeRange = [0 8]
      | sbobj.Groups(17).Name = 'Test Case 17'
      | sbobj.Groups(17).Signals(1).Name = 'DW1'
      | sbobj.Groups(17).Signals(1).XData = [0 4 4 5 5 7 7 8]
      | sbobj.Groups(17).Signals(1).YData = [3 3 4 4 4 4 0 0]
      | sbobj.Groups(17).Signals(2).Name = 'P1W2'
      | sbobj.Groups(17).Signals(2).XData = [0 4 4 5 5 7 7 8]
      | sbobj.Groups(17).Signals(2).YData = [3 3 2 2 4 4 3 3]
      | sbobj.Groups(17).Signals(3).Name = 'O1'
      | sbobj.Groups(17).Signals(3).XData = [0 4 4 5 5 7 7 8]
      | sbobj.Groups(17).Signals(3).YData = [1 1 1 1 1 1 0 0]
      | sbobj.Groups(17).Signals(4).Name = 'O2'
      | sbobj.Groups(17).Signals(4).XData = [0 4 4 5 5 7 7 8]
      | sbobj.Groups(17).Signals(4).YData = [0 0 0 0 0 0 1 1]
      | sbobj.Groups(17).TimeRange = [0 8]
      | sbobj.Groups(18).Name = 'Test Case 18'
      | sbobj.Groups(18).Signals(1).Name = 'DW1'
      | sbobj.Groups(18).Signals(1).XData = [0 4 4 5 5 7 7 8]
      | sbobj.Groups(18).Signals(1).YData = [3 3 4 4 4 4 0 0]
      | sbobj.Groups(18).Signals(2).Name = 'P1W2'
      | sbobj.Groups(18).Signals(2).XData = [0 4 4 5 5 7 7 8]
      | sbobj.Groups(18).Signals(2).YData = [3 3 2 2 1 1 4 4]
      | sbobj.Groups(18).Signals(3).Name = 'O1'
      | sbobj.Groups(18).Signals(3).XData = [0 4 4 5 5 7 7 8]
      | sbobj.Groups(18).Signals(3).YData = [1 1 1 1 1 1 1 1]
      | sbobj.Groups(18).Signals(4).Name = 'O2'
      | sbobj.Groups(18).Signals(4).XData = [0 4 4 5 5 7 7 8]
      | sbobj.Groups(18).Signals(4).YData = [0 0 0 0 0 0 0 0]
      | sbobj.Groups(18).TimeRange = [0 8]
      | sbobj.Groups(19).Name = 'Test Case 19'
      | sbobj.Groups(19).Signals(1).Name = 'DW1'
      | sbobj.Groups(19).Signals(1).XData = [0 4 4 7 7 8]
      | sbobj.Groups(19).Signals(1).YData = [3 3 4 4 2 2]
      | sbobj.Groups(19).Signals(2).Name = 'P1W2'
      | sbobj.Groups(19).Signals(2).XData = [0 4 4 7 7 8]
      | sbobj.Groups(19).Signals(2).YData = [3 3 1 1 2 2]
      | sbobj.Groups(19).Signals(3).Name = 'O1'
      | sbobj.Groups(19).Signals(3).XData = [0 4 4 7 7 8]
      | sbobj.Groups(19).Signals(3).YData = [1 1 0 0 1 1]
      | sbobj.Groups(19).Signals(4).Name = 'O2'
      | sbobj.Groups(19).Signals(4).XData = [0 4 4 7 7 8]
      | sbobj.Groups(19).Signals(4).YData = [0 0 0 0 1 1]
      | sbobj.Groups(19).TimeRange = [0 8]
      | sbobj.Groups(20).Name = 'Test Case 20'
      | sbobj.Groups(20).Signals(1).Name = 'DW1'
      | sbobj.Groups(20).Signals(1).XData = [0 2 2 3 3 4 4 6 6 7]
      | sbobj.Groups(20).Signals(1).YData = [1 1 3 3 2 2 3 3 4 4]
      | sbobj.Groups(20).Signals(2).Name = 'P1W2'
      | sbobj.Groups(20).Signals(2).XData = [0 2 2 3 3 4 4 6 6 7]
      | sbobj.Groups(20).Signals(2).YData = [4 4 0 0 0 0 0 0 0 0]
      | sbobj.Groups(20).Signals(3).Name = 'O1'
      | sbobj.Groups(20).Signals(3).XData = [0 2 2 3 3 4 4 6 6 7]
      | sbobj.Groups(20).Signals(3).YData = [1 1 1 1 0 0 0 0 0 0]
      | sbobj.Groups(20).Signals(4).Name = 'O2'
      | sbobj.Groups(20).Signals(4).XData = [0 2 2 3 3 4 4 6 6 7]
      | sbobj.Groups(20).Signals(4).YData = [0 0 1 1 0 0 0 0 0 0]
      | sbobj.Groups(20).TimeRange = [0 7]
      | sbobj.Groups(21).Name = 'Test Case 21'
      | sbobj.Groups(21).Signals(1).Name = 'DW1'
      | sbobj.Groups(21).Signals(1).XData = [0 2 2 3 3 4 4 6 6 7]
      | sbobj.Groups(21).Signals(1).YData = [1 1 3 3 2 2 4 4 1 1]
      | sbobj.Groups(21).Signals(2).Name = 'P1W2'
      | sbobj.Groups(21).Signals(2).XData = [0 2 2 3 3 4 4 6 6 7]
      | sbobj.Groups(21).Signals(2).YData = [4 4 0 0 0 0 0 0 2 2]
      | sbobj.Groups(21).Signals(3).Name = 'O1'
      | sbobj.Groups(21).Signals(3).XData = [0 2 2 3 3 4 4 6 6 7]
      | sbobj.Groups(21).Signals(3).YData = [1 1 1 1 0 0 0 0 0 0]
      | sbobj.Groups(21).Signals(4).Name = 'O2'
      | sbobj.Groups(21).Signals(4).XData = [0 2 2 3 3 4 4 6 6 7]
      | sbobj.Groups(21).Signals(4).YData = [0 0 1 1 0 0 0 0 0 0]
      | sbobj.Groups(21).TimeRange = [0 7]
      | sbobj.Groups(22).Name = 'Test Case 22'
      | sbobj.Groups(22).Signals(1).Name = 'DW1'
      | sbobj.Groups(22).Signals(1).XData = [0 2 2 3 3 4 4 6 6 7]
      | sbobj.Groups(22).Signals(1).YData = [1 1 3 3 2 2 1 1 4 4]
      | sbobj.Groups(22).Signals(2).Name = 'P1W2'
      | sbobj.Groups(22).Signals(2).XData = [0 2 2 3 3 4 4 6 6 7]
      | sbobj.Groups(22).Signals(2).YData = [4 4 0 0 0 0 0 0 4 4]
      | sbobj.Groups(22).Signals(3).Name = 'O1'
      | sbobj.Groups(22).Signals(3).XData = [0 2 2 3 3 4 4 6 6 7]
      | sbobj.Groups(22).Signals(3).YData = [1 1 1 1 0 0 0 0 0 0]
      | sbobj.Groups(22).Signals(4).Name = 'O2'
      | sbobj.Groups(22).Signals(4).XData = [0 2 2 3 3 4 4 6 6 7]
      | sbobj.Groups(22).Signals(4).YData = [0 0 1 1 0 0 0 0 0 0]
      | sbobj.Groups(22).TimeRange = [0 7]
      | sbobj.Groups(23).Name = 'Test Case 23'
      | sbobj.Groups(23).Signals(1).Name = 'DW1'
      | sbobj.Groups(23).Signals(1).XData = [0 2 2 4 4 5 5 7 7 8]
      | sbobj.Groups(23).Signals(1).YData = [1 1 2 2 0 0 0 0 1 1]
      | sbobj.Groups(23).Signals(2).Name = 'P1W2'
      | sbobj.Groups(23).Signals(2).XData = [0 2 2 4 4 5 5 7 7 8]
      | sbobj.Groups(23).Signals(2).YData = [4 4 3 3 1 1 0 0 2 2]
      | sbobj.Groups(23).Signals(3).Name = 'O1'
      | sbobj.Groups(23).Signals(3).XData = [0 2 2 4 4 5 5 7 7 8]
      | sbobj.Groups(23).Signals(3).YData = [1 1 1 1 1 1 1 1 0 0]
      | sbobj.Groups(23).Signals(4).Name = 'O2'
      | sbobj.Groups(23).Signals(4).XData = [0 2 2 4 4 5 5 7 7 8]
      | sbobj.Groups(23).Signals(4).YData = [0 0 1 1 1 1 0 0 1 1]
      | sbobj.Groups(23).TimeRange = [0 8]
      | sbobj.Groups(24).Name = 'Test Case 24'
      | sbobj.Groups(24).Signals(1).Name = 'DW1'
      | sbobj.Groups(24).Signals(1).XData = [0 2 2 4 4 5 5 7 7 8]
      | sbobj.Groups(24).Signals(1).YData = [1 1 2 2 3 3 3 3 1 1]
      | sbobj.Groups(24).Signals(2).Name = 'P1W2'
      | sbobj.Groups(24).Signals(2).XData = [0 2 2 4 4 5 5 7 7 8]
      | sbobj.Groups(24).Signals(2).YData = [4 4 3 3 1 1 4 4 1 1]
      | sbobj.Groups(24).Signals(3).Name = 'O1'
      | sbobj.Groups(24).Signals(3).XData = [0 2 2 4 4 5 5 7 7 8]
      | sbobj.Groups(24).Signals(3).YData = [1 1 1 1 1 1 1 1 1 1]
      | sbobj.Groups(24).Signals(4).Name = 'O2'
      | sbobj.Groups(24).Signals(4).XData = [0 2 2 4 4 5 5 7 7 8]
      | sbobj.Groups(24).Signals(4).YData = [0 0 1 1 0 0 0 0 0 0]
      | sbobj.Groups(24).TimeRange = [0 8]
      | sbobj.Groups(25).Name = 'Test Case 25'
      | sbobj.Groups(25).Signals(1).Name = 'DW1'
      | sbobj.Groups(25).Signals(1).XData = [0 4 4 5 5 7 7 8]
      | sbobj.Groups(25).Signals(1).YData = [1 1 3 3 3 3 4 4]
      | sbobj.Groups(25).Signals(2).Name = 'P1W2'
      | sbobj.Groups(25).Signals(2).XData = [0 4 4 5 5 7 7 8]
      | sbobj.Groups(25).Signals(2).YData = [4 4 1 1 3 3 4 4]
      | sbobj.Groups(25).Signals(3).Name = 'O1'
      | sbobj.Groups(25).Signals(3).XData = [0 4 4 5 5 7 7 8]
      | sbobj.Groups(25).Signals(3).YData = [1 1 1 1 1 1 1 1]
      | sbobj.Groups(25).Signals(4).Name = 'O2'
      | sbobj.Groups(25).Signals(4).XData = [0 4 4 5 5 7 7 8]
      | sbobj.Groups(25).Signals(4).YData = [0 0 1 1 0 0 1 1]
      | sbobj.Groups(25).TimeRange = [0 8]
      | sbobj.Groups(26).Name = 'Test Case 26'
      | sbobj.Groups(26).Signals(1).Name = 'DW1'
      | sbobj.Groups(26).Signals(1).XData = [0 4 4 5 5 7 7 8]
      | sbobj.Groups(26).Signals(1).YData = [1 1 3 3 3 3 0 0]
      | sbobj.Groups(26).Signals(2).Name = 'P1W2'
      | sbobj.Groups(26).Signals(2).XData = [0 4 4 5 5 7 7 8]
      | sbobj.Groups(26).Signals(2).YData = [4 4 1 1 2 2 0 0]
      | sbobj.Groups(26).Signals(3).Name = 'O1'
      | sbobj.Groups(26).Signals(3).XData = [0 4 4 5 5 7 7 8]
      | sbobj.Groups(26).Signals(3).YData = [1 1 1 1 1 1 0 0]
      | sbobj.Groups(26).Signals(4).Name = 'O2'
      | sbobj.Groups(26).Signals(4).XData = [0 4 4 5 5 7 7 8]
      | sbobj.Groups(26).Signals(4).YData = [0 0 1 1 0 0 0 0]
      | sbobj.Groups(26).TimeRange = [0 8]
  DW1 : Outport  Tag=STV Outport
  P1W2 : Outport  Tag=STV Outport  Port=2
  O1 : Outport  Tag=STV Outport  Port=3
  O2 : Outport  Tag=STV Outport  Port=4
  wires:
  Demux/4 -> O2/1
  Demux/3 -> O1/1
  Demux/2 -> P1W2/1
  Demux/1 -> DW1/1
  FromWs/1 -> Demux/1

== system c00001M_harness/M001 ==
  DW1 : Inport  OutMin=0  OutMax=4  OutDataTypeStr=int8
  P1W2 : Inport  Port=2  OutMin=0  OutMax=4  OutDataTypeStr=int8
  O1 : Inport  Port=3  OutDataTypeStr=boolean
  O2 : Inport  Port=4  OutDataTypeStr=boolean
  Cyber : Subsystem
  M : Memory
  M1 : Memory
  Physical : Subsystem
  S1 : Subsystem
  S2 : Subsystem
  W1Pos : Outport
  W2Pos : Outport  Port=2
  wires:
  S1/1(SensorOut) -> M/1
  Physical/1(W1) -> W1Pos/1, S1/1(PhyMeasure)
  O2/1 -> Cyber/6(OW2)
  O1/1 -> Cyber/5(OW1)
  Cyber/1(W1) -> Physical/1(InW1)
  Cyber/2(W2) -> Physical/2(InW2)
  P1W2/1 -> Cyber/4(P1W2)
  M1/1 -> Cyber/2(PosW2)
  M/1 -> Cyber/1(PosW1)
  DW1/1 -> Cyber/3(DW1)
  Physical/2(W2) -> W2Pos/1, S2/1(PhyMeasure)
  S2/1(SensorOut) -> M1/1

== system c00001M_harness/M002 ==
  DW1 : Inport  OutMin=0  OutMax=4  OutDataTypeStr=int8
  P1W2 : Inport  Port=2  OutMin=0  OutMax=4  OutDataTypeStr=int8
  O1 : Inport  Port=3  OutDataTypeStr=boolean
  O2 : Inport  Port=4  OutDataTypeStr=boolean
  Cyber : Subsystem
  M : Memory
  M1 : Memory
  Physical : Subsystem
  S1 : Subsystem
  S2 : Subsystem
  W1Pos : Outport
  W2Pos : Outport  Port=2
  wires:
  S2/1(SensorOut) -> M1/1
  Physical/2(W2) -> S2/1(PhyMeasure), W2Pos/1
  DW1/1 -> Cyber/3(DW1)
  M/1 -> Cyber/1(PosW1)
  M1/1 -> Cyber/2(PosW2)
  P1W2/1 -> Cyber/4(P1W2)
  Cyber/2(W2) -> Physical/2(InW2)
  Cyber/1(W1) -> Physical/1(InW1)
  O1/1 -> Cyber/5(OW1)
  O2/1 -> Cyber/6(OW2)
  Physical/1(W1) -> S1/1(PhyMeasure), W1Pos/1
  S1/1(SensorOut) -> M/1

== system c00001M_harness/M003 ==
  DW1 : Inport  OutMin=0  OutMax=4  OutDataTypeStr=int8
  P1W2 : Inport  Port=2  OutMin=0  OutMax=4  OutDataTypeStr=int8
  O1 : Inport  Port=3  OutDataTypeStr=boolean
  O2 : Inport  Port=4  OutDataTypeStr=boolean
  Cyber : Subsystem
  M : Memory
  M1 : Memory
  Physical : Subsystem
  S1 : Subsystem
  S2 : Subsystem
  W1Pos : Outport
  W2Pos : Outport  Port=2
  wires:
  S2/1(SensorOut) -> M1/1
  Physical/2(W2) -> S2/1(PhyMeasure), W2Pos/1
  DW1/1 -> Cyber/3(DW1)
  M/1 -> Cyber/1(PosW1)
  M1/1 -> Cyber/2(PosW2)
  P1W2/1 -> Cyber/4(P1W2)
  Cyber/2(W2) -> Physical/2(InW2)
  Cyber/1(W1) -> Physical/1(InW1)
  O1/1 -> Cyber/5(OW1)
  O2/1 -> Cyber/6(OW2)
  Physical/1(W1) -> S1/1(PhyMeasure), W1Pos/1
  S1/1(SensorOut) -> M/1

== system c00001M_harness/M004 ==
  DW1 : Inport  OutMin=0  OutMax=4  OutDataTypeStr=int8
  P1W2 : Inport  Port=2  OutMin=0  OutMax=4  OutDataTypeStr=int8
  O1 : Inport  Port=3  OutDataTypeStr=boolean
  O2 : Inport  Port=4  OutDataTypeStr=boolean
  Cyber : Subsystem
  M : Memory
  M1 : Memory
  Physical : Subsystem
  S1 : Subsystem
  S2 : Subsystem
  W1Pos : Outport
  W2Pos : Outport  Port=2
  wires:
  S2/1(SensorOut) -> M1/1
  Physical/2(W2) -> S2/1(PhyMeasure), W2Pos/1
  DW1/1 -> Cyber/3(DW1)
  M/1 -> Cyber/1(PosW1)
  M1/1 -> Cyber/2(PosW2)
  P1W2/1 -> Cyber/4(P1W2)
  Cyber/2(W2) -> Physical/2(InW2)
  Cyber/1(W1) -> Physical/1(InW1)
  O1/1 -> Cyber/5(OW1)
  O2/1 -> Cyber/6(OW2)
  Physical/1(W1) -> S1/1(PhyMeasure), W1Pos/1
  S1/1(SensorOut) -> M/1

== system c00001M_harness/M011 ==
  DW1 : Inport  OutMin=0  OutMax=4  OutDataTypeStr=int8
  P1W2 : Inport  Port=2  OutMin=0  OutMax=4  OutDataTypeStr=int8
  O1 : Inport  Port=3  OutDataTypeStr=boolean
  O2 : Inport  Port=4  OutDataTypeStr=boolean
  Cyber : Subsystem
  M : Memory
  M1 : Memory
  Physical : Subsystem
  S1 : Subsystem
  S2 : Subsystem
  W1Pos : Outport
  W2Pos : Outport  Port=2
  wires:
  S2/1(SensorOut) -> M1/1
  Physical/2(W2) -> S2/1(PhyMeasure), W2Pos/1
  DW1/1 -> Cyber/3(DW1)
  M/1 -> Cyber/1(PosW1)
  M1/1 -> Cyber/2(PosW2)
  P1W2/1 -> Cyber/4(P1W2)
  Cyber/2(W2) -> Physical/2(InW2)
  Cyber/1(W1) -> Physical/1(InW1)
  O1/1 -> Cyber/5(OW1)
  O2/1 -> Cyber/6(OW2)
  Physical/1(W1) -> S1/1(PhyMeasure), W1Pos/1
  S1/1(SensorOut) -> M/1

== system c00001M_harness/M012 ==
  DW1 : Inport  OutMin=0  OutMax=4  OutDataTypeStr=int8
  P1W2 : Inport  Port=2  OutMin=0  OutMax=4  OutDataTypeStr=int8
  O1 : Inport  Port=3  OutDataTypeStr=boolean
  O2 : Inport  Port=4  OutDataTypeStr=boolean
  Cyber : Subsystem
  M : Memory
  M1 : Memory
  Physical : Subsystem
  S1 : Subsystem
  S2 : Subsystem
  W1Pos : Outport
  W2Pos : Outport  Port=2
  wires:
  S2/1(SensorOut) -> M1/1
  Physical/2(W2) -> S2/1(PhyMeasure), W2Pos/1
  DW1/1 -> Cyber/3(DW1)
  M/1 -> Cyber/1(PosW1)
  M1/1 -> Cyber/2(PosW2)
  P1W2/1 -> Cyber/4(P1W2)
  Cyber/2(W2) -> Physical/2(InW2)
  Cyber/1(W1) -> Physical/1(InW1)
  O1/1 -> Cyber/5(OW1)
  O2/1 -> Cyber/6(OW2)
  Physical/1(W1) -> S1/1(PhyMeasure), W1Pos/1
  S1/1(SensorOut) -> M/1

== system c00001M_harness/M015 ==
  DW1 : Inport  OutMin=0  OutMax=4  OutDataTypeStr=int8
  P1W2 : Inport  Port=2  OutMin=0  OutMax=4  OutDataTypeStr=int8
  O1 : Inport  Port=3  OutDataTypeStr=boolean
  O2 : Inport  Port=4  OutDataTypeStr=boolean
  Cyber : Subsystem
  M : Memory
  M1 : Memory
  Physical : Subsystem
  S1 : Subsystem
  S2 : Subsystem
  W1Pos : Outport
  W2Pos : Outport  Port=2
  wires:
  S2/1(SensorOut) -> M1/1
  Physical/2(W2) -> S2/1(PhyMeasure), W2Pos/1
  DW1/1 -> Cyber/3(DW1)
  M/1 -> Cyber/1(PosW1)
  M1/1 -> Cyber/2(PosW2)
  P1W2/1 -> Cyber/4(P1W2)
  Cyber/2(W2) -> Physical/2(InW2)
  Cyber/1(W1) -> Physical/1(InW1)
  O1/1 -> Cyber/5(OW1)
  O2/1 -> Cyber/6(OW2)
  Physical/1(W1) -> S1/1(PhyMeasure), W1Pos/1
  S1/1(SensorOut) -> M/1

== system c00001M_harness/M016 ==
  DW1 : Inport  OutMin=0  OutMax=4  OutDataTypeStr=int8
  P1W2 : Inport  Port=2  OutMin=0  OutMax=4  OutDataTypeStr=int8
  O1 : Inport  Port=3  OutDataTypeStr=boolean
  O2 : Inport  Port=4  OutDataTypeStr=boolean
  Cyber : Subsystem
  M : Memory
  M1 : Memory
  Physical : Subsystem
  S1 : Subsystem
  S2 : Subsystem
  W1Pos : Outport
  W2Pos : Outport  Port=2
  wires:
  S2/1(SensorOut) -> M1/1
  Physical/2(W2) -> S2/1(PhyMeasure), W2Pos/1
  DW1/1 -> Cyber/3(DW1)
  M/1 -> Cyber/1(PosW1)
  M1/1 -> Cyber/2(PosW2)
  P1W2/1 -> Cyber/4(P1W2)
  Cyber/2(W2) -> Physical/2(InW2)
  Cyber/1(W1) -> Physical/1(InW1)
  O1/1 -> Cyber/5(OW1)
  O2/1 -> Cyber/6(OW2)
  Physical/1(W1) -> S1/1(PhyMeasure), W1Pos/1
  S1/1(SensorOut) -> M/1

== system c00001M_harness/M019 ==
  DW1 : Inport  OutMin=0  OutMax=4  OutDataTypeStr=int8
  P1W2 : Inport  Port=2  OutMin=0  OutMax=4  OutDataTypeStr=int8
  O1 : Inport  Port=3  OutDataTypeStr=boolean
  O2 : Inport  Port=4  OutDataTypeStr=boolean
  Cyber : Subsystem
  M : Memory
  M1 : Memory
  Physical : Subsystem
  S1 : Subsystem
  S2 : Subsystem
  W1Pos : Outport
  W2Pos : Outport  Port=2
  wires:
  S2/1(SensorOut) -> M1/1
  Physical/2(W2) -> S2/1(PhyMeasure), W2Pos/1
  DW1/1 -> Cyber/3(DW1)
  M/1 -> Cyber/1(PosW1)
  M1/1 -> Cyber/2(PosW2)
  P1W2/1 -> Cyber/4(P1W2)
  Cyber/2(W2) -> Physical/2(InW2)
  Cyber/1(W1) -> Physical/1(InW1)
  O1/1 -> Cyber/5(OW1)
  O2/1 -> Cyber/6(OW2)
  Physical/1(W1) -> S1/1(PhyMeasure), W1Pos/1
  S1/1(SensorOut) -> M/1

== system c00001M_harness/M020 ==
  DW1 : Inport  OutMin=0  OutMax=4  OutDataTypeStr=int8
  P1W2 : Inport  Port=2  OutMin=0  OutMax=4  OutDataTypeStr=int8
  O1 : Inport  Port=3  OutDataTypeStr=boolean
  O2 : Inport  Port=4  OutDataTypeStr=boolean
  Cyber : Subsystem
  M : Memory
  M1 : Memory
  Physical : Subsystem
  S1 : Subsystem
  S2 : Subsystem
  W1Pos : Outport
  W2Pos : Outport  Port=2
  wires:
  S2/1(SensorOut) -> M1/1
  Physical/2(W2) -> S2/1(PhyMeasure), W2Pos/1
  DW1/1 -> Cyber/3(DW1)
  M/1 -> Cyber/1(PosW1)
  M1/1 -> Cyber/2(PosW2)
  P1W2/1 -> Cyber/4(P1W2)
  Cyber/2(W2) -> Physical/2(InW2)
  Cyber/1(W1) -> Physical/1(InW1)
  O1/1 -> Cyber/5(OW1)
  O2/1 -> Cyber/6(OW2)
  Physical/1(W1) -> S1/1(PhyMeasure), W1Pos/1
  S1/1(SensorOut) -> M/1

== system c00001M_harness/M023 ==
  DW1 : Inport  OutMin=0  OutMax=4  OutDataTypeStr=int8
  P1W2 : Inport  Port=2  OutMin=0  OutMax=4  OutDataTypeStr=int8
  O1 : Inport  Port=3  OutDataTypeStr=boolean
  O2 : Inport  Port=4  OutDataTypeStr=boolean
  Cyber : Subsystem
  M : Memory
  M1 : Memory
  Physical : Subsystem
  S1 : Subsystem
  S2 : Subsystem
  W1Pos : Outport
  W2Pos : Outport  Port=2
  wires:
  S2/1(SensorOut) -> M1/1
  Physical/2(W2) -> S2/1(PhyMeasure), W2Pos/1
  DW1/1 -> Cyber/3(DW1)
  M/1 -> Cyber/1(PosW1)
  M1/1 -> Cyber/2(PosW2)
  P1W2/1 -> Cyber/4(P1W2)
  Cyber/2(W2) -> Physical/2(InW2)
  Cyber/1(W1) -> Physical/1(InW1)
  O1/1 -> Cyber/5(OW1)
  O2/1 -> Cyber/6(OW2)
  Physical/1(W1) -> S1/1(PhyMeasure), W1Pos/1
  S1/1(SensorOut) -> M/1

== system c00001M_harness/M024 ==
  DW1 : Inport  OutMin=0  OutMax=4  OutDataTypeStr=int8
  P1W2 : Inport  Port=2  OutMin=0  OutMax=4  OutDataTypeStr=int8
  O1 : Inport  Port=3  OutDataTypeStr=boolean
  O2 : Inport  Port=4  OutDataTypeStr=boolean
  Cyber : Subsystem
  M : Memory
  M1 : Memory
  Physical : Subsystem
  S1 : Subsystem
  S2 : Subsystem
  W1Pos : Outport
  W2Pos : Outport  Port=2
  wires:
  S2/1(SensorOut) -> M1/1
  Physical/2(W2) -> S2/1(PhyMeasure), W2Pos/1
  DW1/1 -> Cyber/3(DW1)
  M/1 -> Cyber/1(PosW1)
  M1/1 -> Cyber/2(PosW2)
  P1W2/1 -> Cyber/4(P1W2)
  Cyber/2(W2) -> Physical/2(InW2)
  Cyber/1(W1) -> Physical/1(InW1)
  O1/1 -> Cyber/5(OW1)
  O2/1 -> Cyber/6(OW2)
  Physical/1(W1) -> S1/1(PhyMeasure), W1Pos/1
  S1/1(SensorOut) -> M/1

== system c00001M_harness/M027 ==
  DW1 : Inport  OutMin=0  OutMax=4  OutDataTypeStr=int8
  P1W2 : Inport  Port=2  OutMin=0  OutMax=4  OutDataTypeStr=int8
  O1 : Inport  Port=3  OutDataTypeStr=boolean
  O2 : Inport  Port=4  OutDataTypeStr=boolean
  Cyber : Subsystem
  M : Memory
  M1 : Memory
  Physical : Subsystem
  S1 : Subsystem
  S2 : Subsystem
  W1Pos : Outport
  W2Pos : Outport  Port=2
  wires:
  S2/1(SensorOut) -> M1/1
  Physical/2(W2) -> S2/1(PhyMeasure), W2Pos/1
  DW1/1 -> Cyber/3(DW1)
  M/1 -> Cyber/1(PosW1)
  M1/1 -> Cyber/2(PosW2)
  P1W2/1 -> Cyber/4(P1W2)
  Cyber/2(W2) -> Physical/2(InW2)
  Cyber/1(W1) -> Physical/1(InW1)
  O1/1 -> Cyber/5(OW1)
  O2/1 -> Cyber/6(OW2)
  Physical/1(W1) -> S1/1(PhyMeasure), W1Pos/1
  S1/1(SensorOut) -> M/1

== system c00001M_harness/M028 ==
  DW1 : Inport  OutMin=0  OutMax=4  OutDataTypeStr=int8
  P1W2 : Inport  Port=2  OutMin=0  OutMax=4  OutDataTypeStr=int8
  O1 : Inport  Port=3  OutDataTypeStr=boolean
  O2 : Inport  Port=4  OutDataTypeStr=boolean
  Cyber : Subsystem
  M : Memory
  M1 : Memory
  Physical : Subsystem
  S1 : Subsystem
  S2 : Subsystem
  W1Pos : Outport
  W2Pos : Outport  Port=2
  wires:
  S2/1(SensorOut) -> M1/1
  Physical/2(W2) -> S2/1(PhyMeasure), W2Pos/1
  DW1/1 -> Cyber/3(DW1)
  M/1 -> Cyber/1(PosW1)
  M1/1 -> Cyber/2(PosW2)
  P1W2/1 -> Cyber/4(P1W2)
  Cyber/2(W2) -> Physical/2(InW2)
  Cyber/1(W1) -> Physical/1(InW1)
  O1/1 -> Cyber/5(OW1)
  O2/1 -> Cyber/6(OW2)
  Physical/1(W1) -> S1/1(PhyMeasure), W1Pos/1
  S1/1(SensorOut) -> M/1

== system c00001M_harness/M031 ==
  DW1 : Inport  OutMin=0  OutMax=4  OutDataTypeStr=int8
  P1W2 : Inport  Port=2  OutMin=0  OutMax=4  OutDataTypeStr=int8
  O1 : Inport  Port=3  OutDataTypeStr=boolean
  O2 : Inport  Port=4  OutDataTypeStr=boolean
  Cyber : Subsystem
  M : Memory
  M1 : Memory
  Physical : Subsystem
  S1 : Subsystem
  S2 : Subsystem
  W1Pos : Outport
  W2Pos : Outport  Port=2
  wires:
  S2/1(SensorOut) -> M1/1
  Physical/2(W2) -> S2/1(PhyMeasure), W2Pos/1
  DW1/1 -> Cyber/3(DW1)
  M/1 -> Cyber/1(PosW1)
  M1/1 -> Cyber/2(PosW2)
  P1W2/1 -> Cyber/4(P1W2)
  Cyber/2(W2) -> Physical/2(InW2)
  Cyber/1(W1) -> Physical/1(InW1)
  O1/1 -> Cyber/5(OW1)
  O2/1 -> Cyber/6(OW2)
  Physical/1(W1) -> S1/1(PhyMeasure), W1Pos/1
  S1/1(SensorOut) -> M/1

== system c00001M_harness/M032 ==
  DW1 : Inport  OutMin=0  OutMax=4  OutDataTypeStr=int8
  P1W2 : Inport  Port=2  OutMin=0  OutMax=4  OutDataTypeStr=int8
  O1 : Inport  Port=3  OutDataTypeStr=boolean
  O2 : Inport  Port=4  OutDataTypeStr=boolean
  Cyber : Subsystem
  M : Memory
  M1 : Memory
  Physical : Subsystem
  S1 : Subsystem
  S2 : Subsystem
  W1Pos : Outport
  W2Pos : Outport  Port=2
  wires:
  S2/1(SensorOut) -> M1/1
  Physical/2(W2) -> S2/1(PhyMeasure), W2Pos/1
  DW1/1 -> Cyber/3(DW1)
  M/1 -> Cyber/1(PosW1)
  M1/1 -> Cyber/2(PosW2)
  P1W2/1 -> Cyber/4(P1W2)
  Cyber/2(W2) -> Physical/2(InW2)
  Cyber/1(W1) -> Physical/1(InW1)
  O1/1 -> Cyber/5(OW1)
  O2/1 -> Cyber/6(OW2)
  Physical/1(W1) -> S1/1(PhyMeasure), W1Pos/1
  S1/1(SensorOut) -> M/1

== system c00001M_harness/M035 ==
  DW1 : Inport  OutMin=0  OutMax=4  OutDataTypeStr=int8
  P1W2 : Inport  Port=2  OutMin=0  OutMax=4  OutDataTypeStr=int8
  O1 : Inport  Port=3  OutDataTypeStr=boolean
  O2 : Inport  Port=4  OutDataTypeStr=boolean
  Cyber : Subsystem
  M : Memory
  M1 : Memory
  Physical : Subsystem
  S1 : Subsystem
  S2 : Subsystem
  W1Pos : Outport
  W2Pos : Outport  Port=2
  wires:
  S2/1(SensorOut) -> M1/1
  Physical/2(W2) -> S2/1(PhyMeasure), W2Pos/1
  DW1/1 -> Cyber/3(DW1)
  M/1 -> Cyber/1(PosW1)
  M1/1 -> Cyber/2(PosW2)
  P1W2/1 -> Cyber/4(P1W2)
  Cyber/2(W2) -> Physical/2(InW2)
  Cyber/1(W1) -> Physical/1(InW1)
  O1/1 -> Cyber/5(OW1)
  O2/1 -> Cyber/6(OW2)
  Physical/1(W1) -> S1/1(PhyMeasure), W1Pos/1
  S1/1(SensorOut) -> M/1

== system c00001M_harness/M036 ==
  DW1 : Inport  OutMin=0  OutMax=4  OutDataTypeStr=int8
  P1W2 : Inport  Port=2  OutMin=0  OutMax=4  OutDataTypeStr=int8
  O1 : Inport  Port=3  OutDataTypeStr=boolean
  O2 : Inport  Port=4  OutDataTypeStr=boolean
  Cyber : Subsystem
  M : Memory
  M1 : Memory
  Physical : Subsystem
  S1 : Subsystem
  S2 : Subsystem
  W1Pos : Outport
  W2Pos : Outport  Port=2
  wires:
  S2/1(SensorOut) -> M1/1
  Physical/2(W2) -> S2/1(PhyMeasure), W2Pos/1
  DW1/1 -> Cyber/3(DW1)
  M/1 -> Cyber/1(PosW1)
  M1/1 -> Cyber/2(PosW2)
  P1W2/1 -> Cyber/4(P1W2)
  Cyber/2(W2) -> Physical/2(InW2)
  Cyber/1(W1) -> Physical/1(InW1)
  O1/1 -> Cyber/5(OW1)
  O2/1 -> Cyber/6(OW2)
  Physical/1(W1) -> S1/1(PhyMeasure), W1Pos/1
  S1/1(SensorOut) -> M/1

== system c00001M_harness/M039 ==
  DW1 : Inport  OutMin=0  OutMax=4  OutDataTypeStr=int8
  P1W2 : Inport  Port=2  OutMin=0  OutMax=4  OutDataTypeStr=int8
  O1 : Inport  Port=3  OutDataTypeStr=boolean
  O2 : Inport  Port=4  OutDataTypeStr=boolean
  Cyber : Subsystem
  M : Memory
  M1 : Memory
  Physical : Subsystem
  S1 : Subsystem
  S2 : Subsystem
  W1Pos : Outport
  W2Pos : Outport  Port=2
  wires:
  S2/1(SensorOut) -> M1/1
  Physical/2(W2) -> S2/1(PhyMeasure), W2Pos/1
  DW1/1 -> Cyber/3(DW1)
  M/1 -> Cyber/1(PosW1)
  M1/1 -> Cyber/2(PosW2)
  P1W2/1 -> Cyber/4(P1W2)
  Cyber/2(W2) -> Physical/2(InW2)
  Cyber/1(W1) -> Physical/1(InW1)
  O1/1 -> Cyber/5(OW1)
  O2/1 -> Cyber/6(OW2)
  Physical/1(W1) -> S1/1(PhyMeasure), W1Pos/1
  S1/1(SensorOut) -> M/1

== system c00001M_harness/M040 ==
  DW1 : Inport  OutMin=0  OutMax=4  OutDataTypeStr=int8
  P1W2 : Inport  Port=2  OutMin=0  OutMax=4  OutDataTypeStr=int8
  O1 : Inport  Port=3  OutDataTypeStr=boolean
  O2 : Inport  Port=4  OutDataTypeStr=boolean
  Cyber : Subsystem
  M : Memory
  M1 : Memory
  Physical : Subsystem
  S1 : Subsystem
  S2 : Subsystem
  W1Pos : Outport
  W2Pos : Outport  Port=2
  wires:
  S2/1(SensorOut) -> M1/1
  Physical/2(W2) -> S2/1(PhyMeasure), W2Pos/1
  DW1/1 -> Cyber/3(DW1)
  M/1 -> Cyber/1(PosW1)
  M1/1 -> Cyber/2(PosW2)
  P1W2/1 -> Cyber/4(P1W2)
  Cyber/2(W2) -> Physical/2(InW2)
  Cyber/1(W1) -> Physical/1(InW1)
  O1/1 -> Cyber/5(OW1)
  O2/1 -> Cyber/6(OW2)
  Physical/1(W1) -> S1/1(PhyMeasure), W1Pos/1
  S1/1(SensorOut) -> M/1

== system c00001M_harness/M043 ==
  DW1 : Inport  OutMin=0  OutMax=4  OutDataTypeStr=int8
  P1W2 : Inport  Port=2  OutMin=0  OutMax=4  OutDataTypeStr=int8
  O1 : Inport  Port=3  OutDataTypeStr=boolean
  O2 : Inport  Port=4  OutDataTypeStr=boolean
  Cyber : Subsystem
  M : Memory
  M1 : Memory
  Physical : Subsystem
  S1 : Subsystem
  S2 : Subsystem
  W1Pos : Outport
  W2Pos : Outport  Port=2
  wires:
  S2/1(SensorOut) -> M1/1
  Physical/2(W2) -> S2/1(PhyMeasure), W2Pos/1
  DW1/1 -> Cyber/3(DW1)
  M/1 -> Cyber/1(PosW1)
  M1/1 -> Cyber/2(PosW2)
  P1W2/1 -> Cyber/4(P1W2)
  Cyber/2(W2) -> Physical/2(InW2)
  Cyber/1(W1) -> Physical/1(InW1)
  O1/1 -> Cyber/5(OW1)
  O2/1 -> Cyber/6(OW2)
  Physical/1(W1) -> S1/1(PhyMeasure), W1Pos/1
  S1/1(SensorOut) -> M/1

== system c00001M_harness/M044 ==
  DW1 : Inport  OutMin=0  OutMax=4  OutDataTypeStr=int8
  P1W2 : Inport  Port=2  OutMin=0  OutMax=4  OutDataTypeStr=int8
  O1 : Inport  Port=3  OutDataTypeStr=boolean
  O2 : Inport  Port=4  OutDataTypeStr=boolean
  Cyber : Subsystem
  M : Memory
  M1 : Memory
  Physical : Subsystem
  S1 : Subsystem
  S2 : Subsystem
  W1Pos : Outport
  W2Pos : Outport  Port=2
  wires:
  S2/1(SensorOut) -> M1/1
  Physical/2(W2) -> S2/1(PhyMeasure), W2Pos/1
  DW1/1 -> Cyber/3(DW1)
  M/1 -> Cyber/1(PosW1)
  M1/1 -> Cyber/2(PosW2)
  P1W2/1 -> Cyber/4(P1W2)
  Cyber/2(W2) -> Physical/2(InW2)
  Cyber/1(W1) -> Physical/1(InW1)
  O1/1 -> Cyber/5(OW1)
  O2/1 -> Cyber/6(OW2)
  Physical/1(W1) -> S1/1(PhyMeasure), W1Pos/1
  S1/1(SensorOut) -> M/1

== system c00001M_harness/M047 ==
  DW1 : Inport  OutMin=0  OutMax=4  OutDataTypeStr=int8
  P1W2 : Inport  Port=2  OutMin=0  OutMax=4  OutDataTypeStr=int8
  O1 : Inport  Port=3  OutDataTypeStr=boolean
  O2 : Inport  Port=4  OutDataTypeStr=boolean
  Cyber : Subsystem
  M : Memory
  M1 : Memory
  Physical : Subsystem
  S1 : Subsystem
  S2 : Subsystem
  W1Pos : Outport
  W2Pos : Outport  Port=2
  wires:
  S2/1(SensorOut) -> M1/1
  Physical/2(W2) -> S2/1(PhyMeasure), W2Pos/1
  DW1/1 -> Cyber/3(DW1)
  M/1 -> Cyber/1(PosW1)
  M1/1 -> Cyber/2(PosW2)
  P1W2/1 -> Cyber/4(P1W2)
  Cyber/2(W2) -> Physical/2(InW2)
  Cyber/1(W1) -> Physical/1(InW1)
  O1/1 -> Cyber/5(OW1)
  O2/1 -> Cyber/6(OW2)
  Physical/1(W1) -> S1/1(PhyMeasure), W1Pos/1
  S1/1(SensorOut) -> M/1

== system c00001M_harness/M048 ==
  DW1 : Inport  OutMin=0  OutMax=4  OutDataTypeStr=int8
  P1W2 : Inport  Port=2  OutMin=0  OutMax=4  OutDataTypeStr=int8
  O1 : Inport  Port=3  OutDataTypeStr=boolean
  O2 : Inport  Port=4  OutDataTypeStr=boolean
  Cyber : Subsystem
  M : Memory
  M1 : Memory
  Physical : Subsystem
  S1 : Subsystem
  S2 : Subsystem
  W1Pos : Outport
  W2Pos : Outport  Port=2
  wires:
  S2/1(SensorOut) -> M1/1
  Physical/2(W2) -> S2/1(PhyMeasure), W2Pos/1
  DW1/1 -> Cyber/3(DW1)
  M/1 -> Cyber/1(PosW1)
  M1/1 -> Cyber/2(PosW2)
  P1W2/1 -> Cyber/4(P1W2)
  Cyber/2(W2) -> Physical/2(InW2)
  Cyber/1(W1) -> Physical/1(InW1)
  O1/1 -> Cyber/5(OW1)
  O2/1 -> Cyber/6(OW2)
  Physical/1(W1) -> S1/1(PhyMeasure), W1Pos/1
  S1/1(SensorOut) -> M/1

== system c00001M_harness/M051 ==
  DW1 : Inport  OutMin=0  OutMax=4  OutDataTypeStr=int8
  P1W2 : Inport  Port=2  OutMin=0  OutMax=4  OutDataTypeStr=int8
  O1 : Inport  Port=3  OutDataTypeStr=boolean
  O2 : Inport  Port=4  OutDataTypeStr=boolean
  Cyber : Subsystem
  M : Memory
  M1 : Memory
  Physical : Subsystem
  S1 : Subsystem
  S2 : Subsystem
  W1Pos : Outport
  W2Pos : Outport  Port=2
  wires:
  S2/1(SensorOut) -> M1/1
  Physical/2(W2) -> S2/1(PhyMeasure), W2Pos/1
  DW1/1 -> Cyber/3(DW1)
  M/1 -> Cyber/1(PosW1)
  M1/1 -> Cyber/2(PosW2)
  P1W2/1 -> Cyber/4(P1W2)
  Cyber/2(W2) -> Physical/2(InW2)
  Cyber/1(W1) -> Physical/1(InW1)
  O1/1 -> Cyber/5(OW1)
  O2/1 -> Cyber/6(OW2)
  Physical/1(W1) -> S1/1(PhyMeasure), W1Pos/1
  S1/1(SensorOut) -> M/1

== system c00001M_harness/M052 ==
  DW1 : Inport  OutMin=0  OutMax=4  OutDataTypeStr=int8
  P1W2 : Inport  Port=2  OutMin=0  OutMax=4  OutDataTypeStr=int8
  O1 : Inport  Port=3  OutDataTypeStr=boolean
  O2 : Inport  Port=4  OutDataTypeStr=boolean
  Cyber : Subsystem
  M : Memory
  M1 : Memory
  Physical : Subsystem
  S1 : Subsystem
  S2 : Subsystem
  W1Pos : Outport
  W2Pos : Outport  Port=2
  wires:
  S2/1(SensorOut) -> M1/1
  Physical/2(W2) -> S2/1(PhyMeasure), W2Pos/1
  DW1/1 -> Cyber/3(DW1)
  M/1 -> Cyber/1(PosW1)
  M1/1 -> Cyber/2(PosW2)
  P1W2/1 -> Cyber/4(P1W2)
  Cyber/2(W2) -> Physical/2(InW2)
  Cyber/1(W1) -> Physical/1(InW1)
  O1/1 -> Cyber/5(OW1)
  O2/1 -> Cyber/6(OW2)
  Physical/1(W1) -> S1/1(PhyMeasure), W1Pos/1
  S1/1(SensorOut) -> M/1

== system c00001M_harness/M055 ==
  DW1 : Inport  OutMin=0  OutMax=4  OutDataTypeStr=int8
  P1W2 : Inport  Port=2  OutMin=0  OutMax=4  OutDataTypeStr=int8
  O1 : Inport  Port=3  OutDataTypeStr=boolean
  O2 : Inport  Port=4  OutDataTypeStr=boolean
  Cyber : Subsystem
  M : Memory
  M1 : Memory
  Physical : Subsystem
  S1 : Subsystem
  S2 : Subsystem
  W1Pos : Outport
  W2Pos : Outport  Port=2
  wires:
  S2/1(SensorOut) -> M1/1
  Physical/2(W2) -> S2/1(PhyMeasure), W2Pos/1
  DW1/1 -> Cyber/3(DW1)
  M/1 -> Cyber/1(PosW1)
  M1/1 -> Cyber/2(PosW2)
  P1W2/1 -> Cyber/4(P1W2)
  Cyber/2(W2) -> Physical/2(InW2)
  Cyber/1(W1) -> Physical/1(InW1)
  O1/1 -> Cyber/5(OW1)
  O2/1 -> Cyber/6(OW2)
  Physical/1(W1) -> S1/1(PhyMeasure), W1Pos/1
  S1/1(SensorOut) -> M/1

== system c00001M_harness/M056 ==
  DW1 : Inport  OutMin=0  OutMax=4  OutDataTypeStr=int8
  P1W2 : Inport  Port=2  OutMin=0  OutMax=4  OutDataTypeStr=int8
  O1 : Inport  Port=3  OutDataTypeStr=boolean
  O2 : Inport  Port=4  OutDataTypeStr=boolean
  Cyber : Subsystem
  M : Memory
  M1 : Memory
  Physical : Subsystem
  S1 : Subsystem
  S2 : Subsystem
  W1Pos : Outport
  W2Pos : Outport  Port=2
  wires:
  S2/1(SensorOut) -> M1/1
  Physical/2(W2) -> S2/1(PhyMeasure), W2Pos/1
  DW1/1 -> Cyber/3(DW1)
  M/1 -> Cyber/1(PosW1)
  M1/1 -> Cyber/2(PosW2)
  P1W2/1 -> Cyber/4(P1W2)
  Cyber/2(W2) -> Physical/2(InW2)
  Cyber/1(W1) -> Physical/1(InW1)
  O1/1 -> Cyber/5(OW1)
  O2/1 -> Cyber/6(OW2)
  Physical/1(W1) -> S1/1(PhyMeasure), W1Pos/1
  S1/1(SensorOut) -> M/1

== system c00001M_harness/M059 ==
  DW1 : Inport  OutMin=0  OutMax=4  OutDataTypeStr=int8
  P1W2 : Inport  Port=2  OutMin=0  OutMax=4  OutDataTypeStr=int8
  O1 : Inport  Port=3  OutDataTypeStr=boolean
  O2 : Inport  Port=4  OutDataTypeStr=boolean
  Cyber : Subsystem
  M : Memory
  M1 : Memory
  Physical : Subsystem
  S1 : Subsystem
  S2 : Subsystem
  W1Pos : Outport
  W2Pos : Outport  Port=2
  wires:
  S2/1(SensorOut) -> M1/1
  Physical/2(W2) -> S2/1(PhyMeasure), W2Pos/1
  DW1/1 -> Cyber/3(DW1)
  M/1 -> Cyber/1(PosW1)
  M1/1 -> Cyber/2(PosW2)
  P1W2/1 -> Cyber/4(P1W2)
  Cyber/2(W2) -> Physical/2(InW2)
  Cyber/1(W1) -> Physical/1(InW1)
  O1/1 -> Cyber/5(OW1)
  O2/1 -> Cyber/6(OW2)
  Physical/1(W1) -> S1/1(PhyMeasure), W1Pos/1
  S1/1(SensorOut) -> M/1

== system c00001M_harness/M060 ==
  DW1 : Inport  OutMin=0  OutMax=4  OutDataTypeStr=int8
  P1W2 : Inport  Port=2  OutMin=0  OutMax=4  OutDataTypeStr=int8
  O1 : Inport  Port=3  OutDataTypeStr=boolean
  O2 : Inport  Port=4  OutDataTypeStr=boolean
  Cyber : Subsystem
  M : Memory
  M1 : Memory
  Physical : Subsystem
  S1 : Subsystem
  S2 : Subsystem
  W1Pos : Outport
  W2Pos : Outport  Port=2
  wires:
  S2/1(SensorOut) -> M1/1
  Physical/2(W2) -> S2/1(PhyMeasure), W2Pos/1
  DW1/1 -> Cyber/3(DW1)
  M/1 -> Cyber/1(PosW1)
  M1/1 -> Cyber/2(PosW2)
  P1W2/1 -> Cyber/4(P1W2)
  Cyber/2(W2) -> Physical/2(InW2)
  Cyber/1(W1) -> Physical/1(InW1)
  O1/1 -> Cyber/5(OW1)
  O2/1 -> Cyber/6(OW2)
  Physical/1(W1) -> S1/1(PhyMeasure), W1Pos/1
  S1/1(SensorOut) -> M/1

== system c00001M_harness/M063 ==
  DW1 : Inport  OutMin=0  OutMax=4  OutDataTypeStr=int8
  P1W2 : Inport  Port=2  OutMin=0  OutMax=4  OutDataTypeStr=int8
  O1 : Inport  Port=3  OutDataTypeStr=boolean
  O2 : Inport  Port=4  OutDataTypeStr=boolean
  Cyber : Subsystem
  M : Memory
  M1 : Memory
  Physical : Subsystem
  S1 : Subsystem
  S2 : Subsystem
  W1Pos : Outport
  W2Pos : Outport  Port=2
  wires:
  S2/1(SensorOut) -> M1/1
  Physical/2(W2) -> S2/1(PhyMeasure), W2Pos/1
  DW1/1 -> Cyber/3(DW1)
  M/1 -> Cyber/1(PosW1)
  M1/1 -> Cyber/2(PosW2)
  P1W2/1 -> Cyber/4(P1W2)
  Cyber/2(W2) -> Physical/2(InW2)
  Cyber/1(W1) -> Physical/1(InW1)
  O1/1 -> Cyber/5(OW1)
  O2/1 -> Cyber/6(OW2)
  Physical/1(W1) -> S1/1(PhyMeasure), W1Pos/1
  S1/1(SensorOut) -> M/1

== system c00001M_harness/M064 ==
  DW1 : Inport  OutMin=0  OutMax=4  OutDataTypeStr=int8
  P1W2 : Inport  Port=2  OutMin=0  OutMax=4  OutDataTypeStr=int8
  O1 : Inport  Port=3  OutDataTypeStr=boolean
  O2 : Inport  Port=4  OutDataTypeStr=boolean
  Cyber : Subsystem
  M : Memory
  M1 : Memory
  Physical : Subsystem
  S1 : Subsystem
  S2 : Subsystem
  W1Pos : Outport
  W2Pos : Outport  Port=2
  wires:
  S2/1(SensorOut) -> M1/1
  Physical/2(W2) -> S2/1(PhyMeasure), W2Pos/1
  DW1/1 -> Cyber/3(DW1)
  M/1 -> Cyber/1(PosW1)
  M1/1 -> Cyber/2(PosW2)
  P1W2/1 -> Cyber/4(P1W2)
  Cyber/2(W2) -> Physical/2(InW2)
  Cyber/1(W1) -> Physical/1(InW1)
  O1/1 -> Cyber/5(OW1)
  O2/1 -> Cyber/6(OW2)
  Physical/1(W1) -> S1/1(PhyMeasure), W1Pos/1
  S1/1(SensorOut) -> M/1

== system c00001M_harness/M067 ==
  DW1 : Inport  OutMin=0  OutMax=4  OutDataTypeStr=int8
  P1W2 : Inport  Port=2  OutMin=0  OutMax=4  OutDataTypeStr=int8
  O1 : Inport  Port=3  OutDataTypeStr=boolean
  O2 : Inport  Port=4  OutDataTypeStr=boolean
  Cyber : Subsystem
  M : Memory
  M1 : Memory
  Physical : Subsystem
  S1 : Subsystem
  S2 : Subsystem
  W1Pos : Outport
  W2Pos : Outport  Port=2
  wires:
  S2/1(SensorOut) -> M1/1
  Physical/2(W2) -> S2/1(PhyMeasure), W2Pos/1
  DW1/1 -> Cyber/3(DW1)
  M/1 -> Cyber/1(PosW1)
  M1/1 -> Cyber/2(PosW2)
  P1W2/1 -> Cyber/4(P1W2)
  Cyber/2(W2) -> Physical/2(InW2)
  Cyber/1(W1) -> Physical/1(InW1)
  O1/1 -> Cyber/5(OW1)
  O2/1 -> Cyber/6(OW2)
  Physical/1(W1) -> S1/1(PhyMeasure), W1Pos/1
  S1/1(SensorOut) -> M/1

== system c00001M_harness/M068 ==
  DW1 : Inport  OutMin=0  OutMax=4  OutDataTypeStr=int8
  P1W2 : Inport  Port=2  OutMin=0  OutMax=4  OutDataTypeStr=int8
  O1 : Inport  Port=3  OutDataTypeStr=boolean
  O2 : Inport  Port=4  OutDataTypeStr=boolean
  Cyber : Subsystem
  M : Memory
  M1 : Memory
  Physical : Subsystem
  S1 : Subsystem
  S2 : Subsystem
  W1Pos : Outport
  W2Pos : Outport  Port=2
  wires:
  S2/1(SensorOut) -> M1/1
  Physical/2(W2) -> S2/1(PhyMeasure), W2Pos/1
  DW1/1 -> Cyber/3(DW1)
  M/1 -> Cyber/1(PosW1)
  M1/1 -> Cyber/2(PosW2)
  P1W2/1 -> Cyber/4(P1W2)
  Cyber/2(W2) -> Physical/2(InW2)
  Cyber/1(W1) -> Physical/1(InW1)
  O1/1 -> Cyber/5(OW1)
  O2/1 -> Cyber/6(OW2)
  Physical/1(W1) -> S1/1(PhyMeasure), W1Pos/1
  S1/1(SensorOut) -> M/1

== system c00001M_harness/M071 ==
  DW1 : Inport  OutMin=0  OutMax=4  OutDataTypeStr=int8
  P1W2 : Inport  Port=2  OutMin=0  OutMax=4  OutDataTypeStr=int8
  O1 : Inport  Port=3  OutDataTypeStr=boolean
  O2 : Inport  Port=4  OutDataTypeStr=boolean
  Cyber : Subsystem
  M : Memory
  M1 : Memory
  Physical : Subsystem
  S1 : Subsystem
  S2 : Subsystem
  W1Pos : Outport
  W2Pos : Outport  Port=2
  wires:
  S2/1(SensorOut) -> M1/1
  Physical/2(W2) -> S2/1(PhyMeasure), W2Pos/1
  DW1/1 -> Cyber/3(DW1)
  M/1 -> Cyber/1(PosW1)
  M1/1 -> Cyber/2(PosW2)
  P1W2/1 -> Cyber/4(P1W2)
  Cyber/2(W2) -> Physical/2(InW2)
  Cyber/1(W1) -> Physical/1(InW1)
  O1/1 -> Cyber/5(OW1)
  O2/1 -> Cyber/6(OW2)
  Physical/1(W1) -> S1/1(PhyMeasure), W1Pos/1
  S1/1(SensorOut) -> M/1

== system c00001M_harness/M072 ==
  DW1 : Inport  OutMin=0  OutMax=4  OutDataTypeStr=int8
  P1W2 : Inport  Port=2  OutMin=0  OutMax=4  OutDataTypeStr=int8
  O1 : Inport  Port=3  OutDataTypeStr=boolean
  O2 : Inport  Port=4  OutDataTypeStr=boolean
  Cyber : Subsystem
  M : Memory
  M1 : Memory
  Physical : Subsystem
  S1 : Subsystem
  S2 : Subsystem
  W1Pos : Outport
  W2Pos : Outport  Port=2
  wires:
  S2/1(SensorOut) -> M1/1
  Physical/2(W2) -> S2/1(PhyMeasure), W2Pos/1
  DW1/1 -> Cyber/3(DW1)
  M/1 -> Cyber/1(PosW1)
  M1/1 -> Cyber/2(PosW2)
  P1W2/1 -> Cyber/4(P1W2)
  Cyber/2(W2) -> Physical/2(InW2)
  Cyber/1(W1) -> Physical/1(InW1)
  O1/1 -> Cyber/5(OW1)
  O2/1 -> Cyber/6(OW2)
  Physical/1(W1) -> S1/1(PhyMeasure), W1Pos/1
  S1/1(SensorOut) -> M/1

== system c00001M_harness/M075 ==
  DW1 : Inport  OutMin=0  OutMax=4  OutDataTypeStr=int8
  P1W2 : Inport  Port=2  OutMin=0  OutMax=4  OutDataTypeStr=int8
  O1 : Inport  Port=3  OutDataTypeStr=boolean
  O2 : Inport  Port=4  OutDataTypeStr=boolean
  Cyber : Subsystem
  M : Memory
  M1 : Memory
  Physical : Subsystem
  S1 : Subsystem
  S2 : Subsystem
  W1Pos : Outport
  W2Pos : Outport  Port=2
  wires:
  S2/1(SensorOut) -> M1/1
  Physical/2(W2) -> S2/1(PhyMeasure), W2Pos/1
  DW1/1 -> Cyber/3(DW1)
  M/1 -> Cyber/1(PosW1)
  M1/1 -> Cyber/2(PosW2)
  P1W2/1 -> Cyber/4(P1W2)
  Cyber/2(W2) -> Physical/2(InW2)
  Cyber/1(W1) -> Physical/1(InW1)
  O1/1 -> Cyber/5(OW1)
  O2/1 -> Cyber/6(OW2)
  Physical/1(W1) -> S1/1(PhyMeasure), W1Pos/1
  S1/1(SensorOut) -> M/1

== system c00001M_harness/M076 ==
  DW1 : Inport  OutMin=0  OutMax=4  OutDataTypeStr=int8
  P1W2 : Inport  Port=2  OutMin=0  OutMax=4  OutDataTypeStr=int8
  O1 : Inport  Port=3  OutDataTypeStr=boolean
  O2 : Inport  Port=4  OutDataTypeStr=boolean
  Cyber : Subsystem
  M : Memory
  M1 : Memory
  Physical : Subsystem
  S1 : Subsystem
  S2 : Subsystem
  W1Pos : Outport
  W2Pos : Outport  Port=2
  wires:
  S2/1(SensorOut) -> M1/1
  Physical/2(W2) -> S2/1(PhyMeasure), W2Pos/1
  DW1/1 -> Cyber/3(DW1)
  M/1 -> Cyber/1(PosW1)
  M1/1 -> Cyber/2(PosW2)
  P1W2/1 -> Cyber/4(P1W2)
  Cyber/2(W2) -> Physical/2(InW2)
  Cyber/1(W1) -> Physical/1(InW1)
  O1/1 -> Cyber/5(OW1)
  O2/1 -> Cyber/6(OW2)
  Physical/1(W1) -> S1/1(PhyMeasure), W1Pos/1
  S1/1(SensorOut) -> M/1

== system c00001M_harness/M079 ==
  DW1 : Inport  OutMin=0  OutMax=4  OutDataTypeStr=int8
  P1W2 : Inport  Port=2  OutMin=0  OutMax=4  OutDataTypeStr=int8
  O1 : Inport  Port=3  OutDataTypeStr=boolean
  O2 : Inport  Port=4  OutDataTypeStr=boolean
  Cyber : Subsystem
  M : Memory
  M1 : Memory
  Physical : Subsystem
  S1 : Subsystem
  S2 : Subsystem
  W1Pos : Outport
  W2Pos : Outport  Port=2
  wires:
  S2/1(SensorOut) -> M1/1
  Physical/2(W2) -> S2/1(PhyMeasure), W2Pos/1
  DW1/1 -> Cyber/3(DW1)
  M/1 -> Cyber/1(PosW1)
  M1/1 -> Cyber/2(PosW2)
  P1W2/1 -> Cyber/4(P1W2)
  Cyber/2(W2) -> Physical/2(InW2)
  Cyber/1(W1) -> Physical/1(InW1)
  O1/1 -> Cyber/5(OW1)
  O2/1 -> Cyber/6(OW2)
  Physical/1(W1) -> S1/1(PhyMeasure), W1Pos/1
  S1/1(SensorOut) -> M/1

== system c00001M_harness/M080 ==
  DW1 : Inport  OutMin=0  OutMax=4  OutDataTypeStr=int8
  P1W2 : Inport  Port=2  OutMin=0  OutMax=4  OutDataTypeStr=int8
  O1 : Inport  Port=3  OutDataTypeStr=boolean
  O2 : Inport  Port=4  OutDataTypeStr=boolean
  Cyber : Subsystem
  M : Memory
  M1 : Memory
  Physical : Subsystem
  S1 : Subsystem
  S2 : Subsystem
  W1Pos : Outport
  W2Pos : Outport  Port=2
  wires:
  S2/1(SensorOut) -> M1/1
  Physical/2(W2) -> S2/1(PhyMeasure), W2Pos/1
  DW1/1 -> Cyber/3(DW1)
  M/1 -> Cyber/1(PosW1)
  M1/1 -> Cyber/2(PosW2)
  P1W2/1 -> Cyber/4(P1W2)
  Cyber/2(W2) -> Physical/2(InW2)
  Cyber/1(W1) -> Physical/1(InW1)
  O1/1 -> Cyber/5(OW1)
  O2/1 -> Cyber/6(OW2)
  Physical/1(W1) -> S1/1(PhyMeasure), W1Pos/1
  S1/1(SensorOut) -> M/1

== system c00001M_harness/M083 ==
  DW1 : Inport  OutMin=0  OutMax=4  OutDataTypeStr=int8
  P1W2 : Inport  Port=2  OutMin=0  OutMax=4  OutDataTypeStr=int8
  O1 : Inport  Port=3  OutDataTypeStr=boolean
  O2 : Inport  Port=4  OutDataTypeStr=boolean
  Cyber : Subsystem
  M : Memory
  M1 : Memory
  Physical : Subsystem
  S1 : Subsystem
  S2 : Subsystem
  W1Pos : Outport
  W2Pos : Outport  Port=2
  wires:
  S2/1(SensorOut) -> M1/1
  Physical/2(W2) -> S2/1(PhyMeasure), W2Pos/1
  DW1/1 -> Cyber/3(DW1)
  M/1 -> Cyber/1(PosW1)
  M1/1 -> Cyber/2(PosW2)
  P1W2/1 -> Cyber/4(P1W2)
  Cyber/2(W2) -> Physical/2(InW2)
  Cyber/1(W1) -> Physical/1(InW1)
  O1/1 -> Cyber/5(OW1)
  O2/1 -> Cyber/6(OW2)
  Physical/1(W1) -> S1/1(PhyMeasure), W1Pos/1
  S1/1(SensorOut) -> M/1
